simulink model "Project"  (R2017a)
settings: Solver=VariableStepAuto  StartTime=0.0  StopTime=20  FixedStep=0.01  RelTol=1e-3
values from neighbouring files (symbols this model uses):
  b = 2    [initial_condition_and_plots.m]
  c = 4    [initial_condition_and_plots.m]
  C = 2    [initial_condition_and_plots.m]
  Dmax = 3    [initial_condition_and_plots.m]
  init1 = [ -29 -27 pi/6]    [initial_condition_and_plots.m]
  init2 = [ -27 -24 2*pi/3]    [initial_condition_and_plots.m]
  init3 = [ -25 -21 pi/12]    [initial_condition_and_plots.m]
  init4 = [ -23 -19 pi/2]    [initial_condition_and_plots.m]
  init5 = [ -21 -12 5*pi/4]    [initial_condition_and_plots.m]
  K = 4    [initial_condition_and_plots.m]
  K_th = 3    [initial_condition_and_plots.m]
  Kij = 3    [initial_condition_and_plots.m]
  L = 20    [initial_condition_and_plots.m]
  r1k = 3    [initial_condition_and_plots.m]
  r2k = 4    [initial_condition_and_plots.m]
  x1k = 0    [initial_condition_and_plots.m]
  x2k = 15    [initial_condition_and_plots.m]
  y1k = -20    [initial_condition_and_plots.m]
  y2k = -5    [initial_condition_and_plots.m]
  yd = @(i) 4*i-20    [initial_condition_and_plots.m]
(part 1 of 2)
settings Model: Creator=Labis Papakwstas  LastModifiedBy=Labis Papakwstas

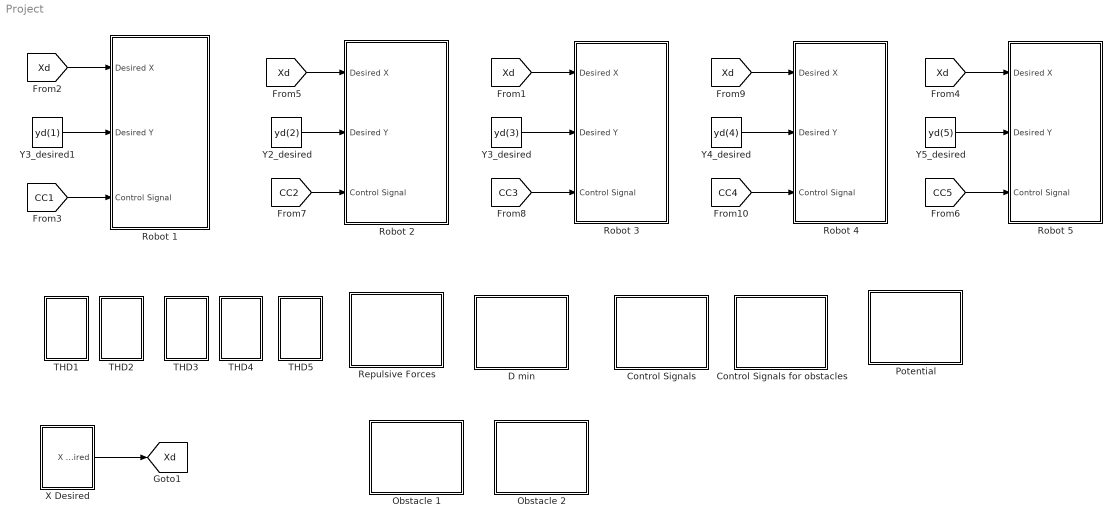
== system Project ==
  "Control Signals " : Subsystem
  Control Signals for obstacles : Subsystem
  D min : Subsystem
  Obstacle 1 : Subsystem
  Obstacle 2 : Subsystem
  Potential : Subsystem
  Repulsive Forces : Subsystem
  "Robot 1 " : Subsystem
  Robot 2 : Subsystem
  Robot 3 : Subsystem
  Robot 4 : Subsystem
  Robot 5 : Subsystem
  "THD1 " : Subsystem
  THD2 : Subsystem
  THD3 : Subsystem
  THD4 : Subsystem
  THD5 : Subsystem
  X Desired : Subsystem
  Y2_desired : Constant  Value=yd(2)
  Y3_desired : Constant  Value=yd(3)
  Y3_desired1 : Constant  Value=yd(1)
  Y4_desired : Constant  Value=yd(4)
  Y5_desired : Constant  Value=yd(5)
  tag scope: Xd=global
  wires:
  [CC3] -> Robot 3/3(Control Signal)
  Y3_desired1/1 -> "Robot 1 "/2("Desired Y ")
  [Xd] -> "Robot 1 "/1(Desired X)
  [CC1] -> "Robot 1 "/3(Control Signal)
  Y2_desired/1 -> Robot 2/2("Desired Y ")
  Y3_desired/1 -> Robot 3/2("Desired Y ")
  [CC2] -> Robot 2/3(Control Signal)
  [Xd] -> Robot 3/1(Desired X)
  X Desired/1(X Desired) -> [Xd]
  [Xd] -> Robot 2/1(Desired X)
  [Xd] -> Robot 5/1(Desired X)
  Y5_desired/1 -> Robot 5/2("Desired Y ")
  [CC5] -> Robot 5/3(Control Signal)
  [CC4] -> Robot 4/3(Control Signal)
  Y4_desired/1 -> Robot 4/2("Desired Y ")
  [Xd] -> Robot 4/1(Desired X)

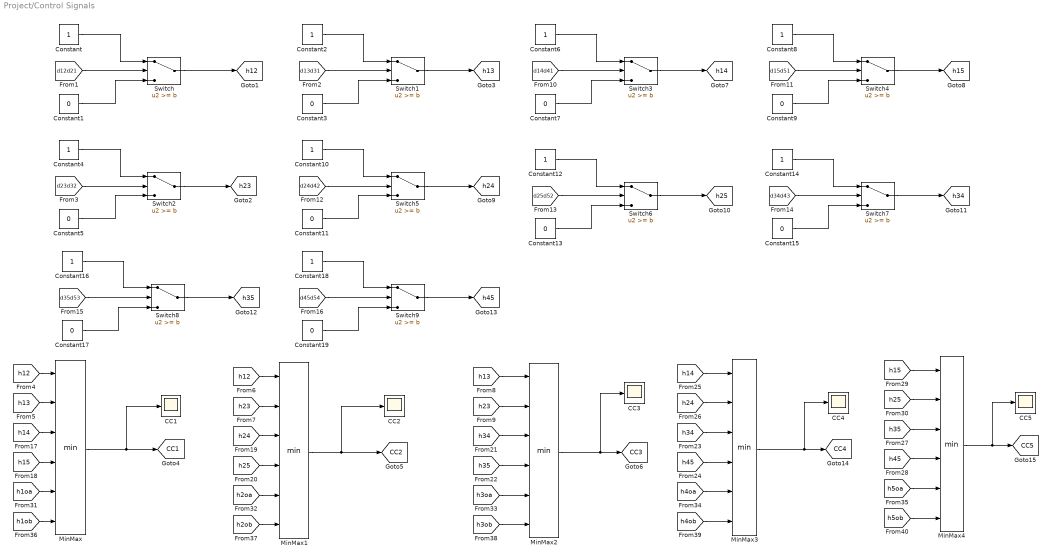
== system Project/Control Signals  ==
  CC1 : Scope
  "CC2 " : Scope
  "CC3 " : Scope
  CC4 : Scope
  CC5 : Scope
  Constant{,2,4,6,8,10,12,14,16,18} (10 alike) : Constant
  Constant{1,3,5,7,9,11,13,15,17,19} (10 alike) : Constant  Value=0
  MinMax{,1..4} (5 alike) : MinMax  Inputs=6
  Switch{,2,5..9} (7 alike) : Switch  Threshold=b
  Switch1 : Switch  Threshold=b  ZeroCross=off
  Switch3 : Switch  Threshold=b  ZeroCross=off
  Switch4 : Switch  Threshold=b  ZeroCross=off
  tag scope: CC1=global, CC2=global, CC3=global, CC4=global, CC5=global, h12=global, h13=global, h14=global, h15=global, h23=global, h24=global, h25=global, h34=global, h35=global, h45=global
  wires:
  [d12d21] -> Switch/2
  Constant/1 -> Switch/1
  Constant1/1 -> Switch/3
  Switch/1 -> [h12]
  [d13d31] -> Switch1/2
  Constant3/1 -> Switch1/3
  Switch1/1 -> [h13]
  Constant2/1 -> Switch1/1
  Switch2/1 -> [h23]
  Constant5/1 -> Switch2/3
  [d23d32] -> Switch2/2
  Constant4/1 -> Switch2/1
  [h12] -> MinMax/1
  [h13] -> MinMax/2
  [h23] -> MinMax1/2
  [h12] -> MinMax1/1
  [h13] -> MinMax2/1
  [h23] -> MinMax2/2
  MinMax1/1 -> "CC2 "/1, [CC2]
  MinMax2/1 -> "CC3 "/1, [CC3]
  MinMax/1 -> CC1/1, [CC1]
  Constant6/1 -> Switch3/1
  Switch3/1 -> [h14]
  Constant7/1 -> Switch3/3
  [d14d41] -> Switch3/2
  [d15d51] -> Switch4/2
  Constant9/1 -> Switch4/3
  Switch4/1 -> [h15]
  Constant8/1 -> Switch4/1
  Constant10/1 -> Switch5/1
  [d24d42] -> Switch5/2
  Constant11/1 -> Switch5/3
  Switch5/1 -> [h24]
  Switch6/1 -> [h25]
  Constant13/1 -> Switch6/3
  [d25d52] -> Switch6/2
  Constant12/1 -> Switch6/1
  Constant14/1 -> Switch7/1
  [d34d43] -> Switch7/2
  Constant15/1 -> Switch7/3
  Switch7/1 -> [h34]
  Switch8/1 -> [h35]
  Constant17/1 -> Switch8/3
  [d35d53] -> Switch8/2
  Constant16/1 -> Switch8/1
  Constant18/1 -> Switch9/1
  [d45d54] -> Switch9/2
  Constant19/1 -> Switch9/3
  Switch9/1 -> [h45]
  [h14] -> MinMax/3
  [h15] -> MinMax/4
  [h24] -> MinMax1/3
  [h25] -> MinMax1/4
  [h34] -> MinMax2/3
  [h35] -> MinMax2/4
  [h45] -> MinMax3/4
  [h34] -> MinMax3/3
  MinMax3/1 -> [CC4], CC4/1
  [h24] -> MinMax3/2
  [h14] -> MinMax3/1
  [h15] -> MinMax4/1
  [h25] -> MinMax4/2
  MinMax4/1 -> [CC5], CC5/1
  [h35] -> MinMax4/3
  [h45] -> MinMax4/4
  [h1oa] -> MinMax/5
  [h2oa] -> MinMax1/5
  [h3oa] -> MinMax2/5
  [h4oa] -> MinMax3/5
  [h5oa] -> MinMax4/5
  [h1ob] -> MinMax/6
  [h2ob] -> MinMax1/6
  [h3ob] -> MinMax2/6
  [h4ob] -> MinMax3/6
  [h5ob] -> MinMax4/6

== system Project/Control Signals for obstacles ==
  Constant{,2,4,6,8,10,12,14,16,18} (10 alike) : Constant
  Constant{1,3,5,7,9,11,13,15,17,19} (10 alike) : Constant  Value=0
  Switch : Switch  Threshold=2  ZeroCross=off
  Switch{1..9} (9 alike) : Switch  Threshold=b
  tag scope: h1oa=global, h1ob=global, h2oa=global, h2ob=global, h3oa=global, h3ob=global, h4oa=global, h4ob=global, h5oa=global, h5ob=global
  wires:
  Switch/1 -> [h1oa]
  Constant1/1 -> Switch/3
  [d1o1] -> Switch/2
  Constant/1 -> Switch/1
  Constant2/1 -> Switch1/1
  [d2o1] -> Switch1/2
  Constant3/1 -> Switch1/3
  Switch1/1 -> [h2oa]
  Switch2/1 -> [h3oa]
  Constant5/1 -> Switch2/3
  [d3o1] -> Switch2/2
  Constant4/1 -> Switch2/1
  Constant6/1 -> Switch3/1
  [d4o1] -> Switch3/2
  Constant7/1 -> Switch3/3
  Switch3/1 -> [h4oa]
  Switch4/1 -> [h5oa]
  Constant9/1 -> Switch4/3
  [d5o1] -> Switch4/2
  Constant8/1 -> Switch4/1
  Constant18/1 -> Switch9/1
  [d5o2] -> Switch9/2
  Constant19/1 -> Switch9/3
  Switch9/1 -> [h5ob]
  Switch8/1 -> [h4ob]
  Constant17/1 -> Switch8/3
  [d4o2] -> Switch8/2
  Constant16/1 -> Switch8/1
  Constant14/1 -> Switch7/1
  [d3o2] -> Switch7/2
  Constant15/1 -> Switch7/3
  Switch7/1 -> [h3ob]
  Switch6/1 -> [h2ob]
  Constant13/1 -> Switch6/3
  [d2o2] -> Switch6/2
  Constant12/1 -> Switch6/1
  Constant10/1 -> Switch5/1
  [d1o2] -> Switch5/2
  Constant11/1 -> Switch5/3
  Switch5/1 -> [h1ob]

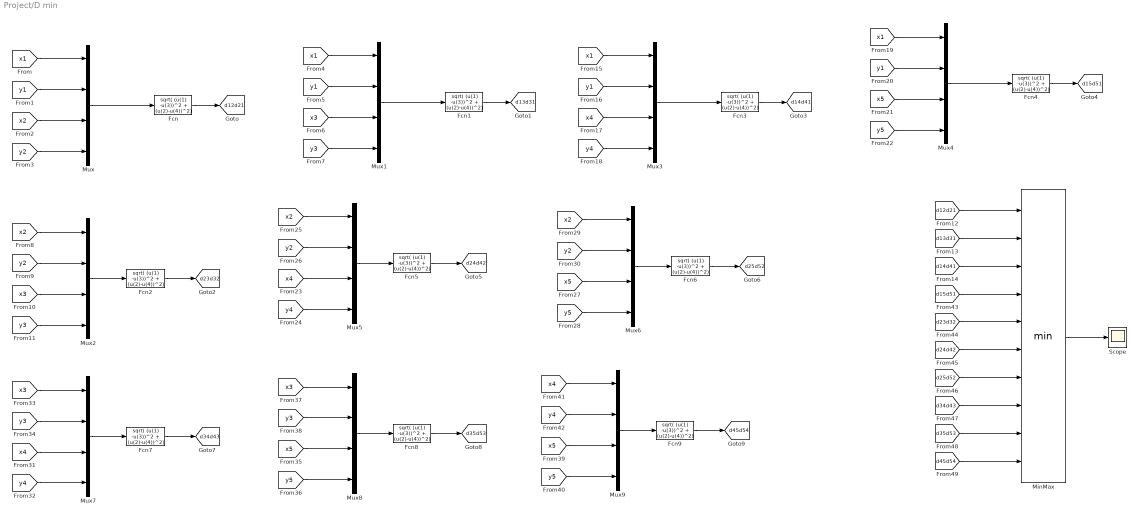
== system Project/D min ==
  Fcn{,1..9} (10 alike) : Fcn  Expr=sqrt( (u(1) -u(3))^2 + (u(2)-u(4))^2)
  MinMax : MinMax  Inputs=10
  Mux{,1..9} (10 alike) : Mux
  Scope : Scope
  tag scope: d12d21=global, d13d31=global, d14d41=global, d15d51=global, d23d32=global, d24d42=global, d25d52=global, d34d43=global, d35d53=global, d45d54=global
  wires:
  [x1] -> Mux/1
  [y1] -> Mux/2
  [x2] -> Mux/3
  [y2] -> Mux/4
  Mux/1 -> Fcn/1
  Mux1/1 -> Fcn1/1
  [y3] -> Mux1/4
  [x3] -> Mux1/3
  [y1] -> Mux1/2
  [x1] -> Mux1/1
  [y2] -> Mux2/2
  [x3] -> Mux2/3
  [x2] -> Mux2/1
  [y3] -> Mux2/4
  Mux2/1 -> Fcn2/1
  Fcn/1 -> [d12d21]
  Fcn1/1 -> [d13d31]
  Fcn2/1 -> [d23d32]
  [d12d21] -> MinMax/1
  [d13d31] -> MinMax/2
  [d14d41] -> MinMax/3
  MinMax/1 -> Scope/1
  Fcn3/1 -> [d14d41]
  [x1] -> Mux3/1
  [y1] -> Mux3/2
  [x4] -> Mux3/3
  [y4] -> Mux3/4
  Mux3/1 -> Fcn3/1
  Mux4/1 -> Fcn4/1
  [y5] -> Mux4/4
  [x5] -> Mux4/3
  [y1] -> Mux4/2
  [x1] -> Mux4/1
  Fcn4/1 -> [d15d51]
  Fcn5/1 -> [d24d42]
  Mux5/1 -> Fcn5/1
  [y4] -> Mux5/4
  [x2] -> Mux5/1
  [x4] -> Mux5/3
  [y2] -> Mux5/2
  [y2] -> Mux6/2
  [x5] -> Mux6/3
  [x2] -> Mux6/1
  [y5] -> Mux6/4
  Mux6/1 -> Fcn6/1
  Fcn6/1 -> [d25d52]
  Fcn7/1 -> [d34d43]
  Mux7/1 -> Fcn7/1
  [y4] -> Mux7/4
  [x3] -> Mux7/1
  [x4] -> Mux7/3
  [y3] -> Mux7/2
  [y3] -> Mux8/2
  [x5] -> Mux8/3
  [x3] -> Mux8/1
  [y5] -> Mux8/4
  Mux8/1 -> Fcn8/1
  Fcn8/1 -> [d35d53]
  Fcn9/1 -> [d45d54]
  Mux9/1 -> Fcn9/1
  [y5] -> Mux9/4
  [x4] -> Mux9/1
  [x5] -> Mux9/3
  [y4] -> Mux9/2
  [d15d51] -> MinMax/4
  [d23d32] -> MinMax/5
  [d24d42] -> MinMax/6
  [d25d52] -> MinMax/7
  [d34d43] -> MinMax/8
  [d35d53] -> MinMax/9
  [d45d54] -> MinMax/10

== system Project/Obstacle 1 ==
  Constant{,3,6,9,12} (5 alike) : Constant  Value=x1k
  Constant{1,4,7,10,13} (5 alike) : Constant  Value=y1k
  Constant{2,5,8,11,14} (5 alike) : Constant  Value=r1k
  Fcn : Fcn  Expr="u(5)*u(1)/(sqrt( (u(1) - u(2))^2 + (u(3) - u(4))^2)) +u(2)* ( 1 - (u(5)/sqrt( ( u(1) - u(2) )^2 + ( u(3) - u(4) )^2) )  )"
  Fcn1 : Fcn  Expr=u(5)*u(3)/(sqrt( (u(1) - u(2))^2 + (u(3) - u(4))^2)) + ( 1 - (u(5)/sqrt( (u(1) - u(2))^2 + (u(3) - u(4))^2)) )*u(4)
  Fcn{2,4,6,8} (4 alike) : Fcn  Expr=u(5)*u(1)/(sqrt( (u(1) - u(2))^2 + (u(3) - u(4))^2)) + ( 1 - u(5)/(sqrt( (u(1) - u(2))^2 + (u(3) - u(4))^2)) )*u(2)
  Fcn{3,5,7,9} (4 alike) : Fcn  Expr=u(5)*u(3)/(sqrt( (u(1) - u(2))^2 + (u(3) - u(4))^2)) + ( 1 - u(5)/(sqrt( (u(1) - u(2))^2 + (u(3) - u(4))^2)) )*u(4)
  Mux{,1..4} (5 alike) : Mux  Inputs=5
  "Obstacle Distance " : Subsystem
  tag scope: x1o1=global, x2o1=global, x3o1=global, x4o1=global, x5o1=global, y1o1=global, y2o1=global, y3o1=global, y4o1=global, y5o1=global
  wires:
  [x1] -> Mux/1
  [y1] -> Mux/3
  Constant2/1 -> Mux/5
  Constant1/1 -> Mux/4
  Constant/1 -> Mux/2
  Mux/1 -> Fcn1/1, Fcn/1
  Fcn/1 -> [x1o1]
  Fcn1/1 -> [y1o1]
  Fcn3/1 -> [y2o1]
  [y2] -> Mux1/3
  [x2] -> Mux1/1
  Constant5/1 -> Mux1/5
  Constant3/1 -> Mux1/2
  Constant4/1 -> Mux1/4
  Fcn2/1 -> [x2o1]
  Mux1/1 -> Fcn3/1, Fcn2/1
  Mux2/1 -> Fcn5/1, Fcn4/1
  Fcn4/1 -> [x3o1]
  Constant6/1 -> Mux2/2
  [x3] -> Mux2/1
  Constant8/1 -> Mux2/5
  [y3] -> Mux2/3
  Constant7/1 -> Mux2/4
  Fcn5/1 -> [y3o1]
  Fcn7/1 -> [y4o1]
  Constant10/1 -> Mux3/4
  [y4] -> Mux3/3
  Constant11/1 -> Mux3/5
  [x4] -> Mux3/1
  Constant9/1 -> Mux3/2
  Fcn6/1 -> [x4o1]
  Mux3/1 -> Fcn6/1, Fcn7/1
  Mux4/1 -> Fcn8/1, Fcn9/1
  Fcn8/1 -> [x5o1]
  Constant13/1 -> Mux4/4
  Constant12/1 -> Mux4/2
  Constant14/1 -> Mux4/5
  [x5] -> Mux4/1
  [y5] -> Mux4/3
  Fcn9/1 -> [y5o1]

== system Project/Obstacle 2 ==
  Constant{,3,6,9,12} (5 alike) : Constant  Value=x2k
  Constant{1,4,7,10,13} (5 alike) : Constant  Value=y2k
  Constant{2,5,8,11,14} (5 alike) : Constant  Value=r2k
  Fcn : Fcn  Expr="u(5)*u(1)/(sqrt( (u(1) - u(2))^2 + (u(3) - u(4))^2)) +u(2)* ( 1 - (u(5)/sqrt( ( u(1) - u(2) )^2 + ( u(3) - u(4) )^2) )  )"
  Fcn1 : Fcn  Expr=u(5)*u(3)/(sqrt( (u(1) - u(2))^2 + (u(3) - u(4))^2)) + ( 1 - (u(5)/sqrt( (u(1) - u(2))^2 + (u(3) - u(4))^2)) )*u(4)
  Fcn{2,4,6,8} (4 alike) : Fcn  Expr=u(5)*u(1)/(sqrt( (u(1) - u(2))^2 + (u(3) - u(4))^2)) + ( 1 - u(5)/(sqrt( (u(1) - u(2))^2 + (u(3) - u(4))^2)) )*u(2)
  Fcn{3,5,7,9} (4 alike) : Fcn  Expr=u(5)*u(3)/(sqrt( (u(1) - u(2))^2 + (u(3) - u(4))^2)) + ( 1 - u(5)/(sqrt( (u(1) - u(2))^2 + (u(3) - u(4))^2)) )*u(4)
  Mux{,1..4} (5 alike) : Mux  Inputs=5
  "Obstacle Distance " : Subsystem
  tag scope: x1o2=global, x2o2=global, x3o2=global, x4o2=global, x5o2=global, y1o2=global, y2o2=global, y3o2=global, y4o2=global, y5o2=global
  wires:
  Fcn9/1 -> [y5o2]
  [y5] -> Mux4/3
  [x5] -> Mux4/1
  Constant14/1 -> Mux4/5
  Constant12/1 -> Mux4/2
  Constant13/1 -> Mux4/4
  Fcn8/1 -> [x5o2]
  Mux4/1 -> Fcn9/1, Fcn8/1
  Mux3/1 -> Fcn7/1, Fcn6/1
  Fcn6/1 -> [x4o2]
  Constant9/1 -> Mux3/2
  [x4] -> Mux3/1
  Constant11/1 -> Mux3/5
  [y4] -> Mux3/3
  Constant10/1 -> Mux3/4
  Fcn7/1 -> [y4o2]
  Fcn5/1 -> [y3o2]
  Constant7/1 -> Mux2/4
  [y3] -> Mux2/3
  Constant8/1 -> Mux2/5
  [x3] -> Mux2/1
  Constant6/1 -> Mux2/2
  Fcn4/1 -> [x3o2]
  Mux2/1 -> Fcn4/1, Fcn5/1
  Mux1/1 -> Fcn2/1, Fcn3/1
  Fcn2/1 -> [x2o2]
  Constant4/1 -> Mux1/4
  Constant3/1 -> Mux1/2
  Constant5/1 -> Mux1/5
  [x2] -> Mux1/1
  [y2] -> Mux1/3
  Fcn3/1 -> [y2o2]
  Fcn1/1 -> [y1o2]
  Fcn/1 -> [x1o2]
  Mux/1 -> Fcn/1, Fcn1/1
  Constant/1 -> Mux/2
  Constant1/1 -> Mux/4
  Constant2/1 -> Mux/5
  [y1] -> Mux/3
  [x1] -> Mux/1

== system Project/Potential ==
  Sum : Sum  Inputs=|+++++
  VA1 : Subsystem
  VA2 : Subsystem
  VA3 : Subsystem
  VA4 : Subsystem
  VA5 : Subsystem
  Va : Scope
  tag scope: Va1=global, Va2=global, Va3=global, Va4=global, Va5=global
  wires:
  VA1/1(Vi) -> [Va1]
  VA2/1(Vi) -> [Va2]
  [Va1] -> Sum/1
  [Va2] -> Sum/2
  [Va3] -> Sum/3
  Sum/1 -> Va/1
  VA3/1(Vi) -> [Va3]
  VA4/1(Vi) -> [Va4]
  VA5/1(Vi) -> [Va5]
  [Va5] -> Sum/5
  [Va4] -> Sum/4

== system Project/Repulsive Forces ==
  Forces Robot1 : Subsystem
  Forces Robot2 : Subsystem
  Forces Robot3 : Subsystem
  Forces Robot4 : Subsystem
  Forces Robot5 : Subsystem
  tag scope: F1x=global, F1y=global, F2x=global, F2y=global, F3x=global, F3y=global, F4x=global, F4y=global, F5x=global, F5y=global
  wires:
  Forces Robot3/1(Fx) -> [F3x]
  Forces Robot3/2(Fy) -> [F3y]
  Forces Robot4/2(Fy) -> [F4y]
  Forces Robot4/1(Fx) -> [F4x]
  Forces Robot5/1(Fx) -> [F5x]
  Forces Robot5/2(Fy) -> [F5y]
  Forces Robot1/1(Fx) -> [F1x]
  Forces Robot1/2(Fy) -> [F1y]
  Forces Robot2/1(Fx) -> [F2x]
  Forces Robot2/2(Fy) -> [F2y]

== system Project/Robot 1  ==
  Desired X : Inport
  "Desired Y " : Inport  Port=2
  Control Signal : Inport  Port=3
  Fcn1 : Fcn  Expr=sqrt( u(1) ^2 + u(2)^2)
  Mux1 : Mux  Inputs=2
  TH1 : Scope
  Tracking Control : Subsystem
  U1 : Scope
  V1 : Scope
  X1 : Scope
  Y1 : Scope
  tag scope: th1=global, x1=global, y1=global
  wires:
  [th1] -> Tracking Control/5(TH1)
  [y1] -> Tracking Control/3(Y1)
  [x1] -> Tracking Control/1(X1)
  Tracking Control/5("U ") -> U1/1
  Tracking Control/4(V) -> V1/1
  Tracking Control/3("TH ") -> TH1/1, [th1]
  Tracking Control/2(Y) -> Y1/1, [y1]
  Tracking Control/1(X) -> X1/1, [x1]
  "Desired Y "/1 -> Tracking Control/4(Yd)
  Desired X/1 -> Tracking Control/2(Xd)
  [F1x] -> Mux1/2
  Mux1/1 -> Fcn1/1
  [F1y] -> Mux1/1
  Fcn1/1 -> Tracking Control/7(Dc)
  Control Signal/1 -> Tracking Control/8(CC)
  [thd1] -> Tracking Control/6(THc)

== system Project/Robot 2 ==
  Desired X : Inport
  "Desired Y " : Inport  Port=2
  Control Signal : Inport  Port=3
  Fcn1 : Fcn  Expr=sqrt( u(1) ^2 + u(2)^2)
  Mux1 : Mux  Inputs=2
  TH2 : Scope
  Tracking Control1 : Subsystem
  U2 : Scope
  V2 : Scope
  X2 : Scope
  Y2 : Scope
  tag scope: th2=global, x2=global, y2=global
  wires:
  Fcn1/1 -> Tracking Control1/7(Dc)
  Control Signal/1 -> Tracking Control1/8(CC)
  Tracking Control1/4(V) -> V2/1
  Tracking Control1/5("U ") -> U2/1
  Mux1/1 -> Fcn1/1
  [thd2] -> Tracking Control1/6(THc)
  [F2x] -> Mux1/2
  Desired X/1 -> Tracking Control1/2(Xd)
  [th2] -> Tracking Control1/5(TH1)
  [x2] -> Tracking Control1/1(X1)
  "Desired Y "/1 -> Tracking Control1/4(Yd)
  Tracking Control1/2(Y) -> Y2/1, [y2]
  Tracking Control1/1(X) -> X2/1, [x2]
  Tracking Control1/3("TH ") -> TH2/1, [th2]
  [F2y] -> Mux1/1
  [y2] -> Tracking Control1/3(Y1)

== system Project/Robot 3 ==
  Desired X : Inport
  "Desired Y " : Inport  Port=2
  Control Signal : Inport  Port=3
  Fcn1 : Fcn  Expr=sqrt( u(1) ^2 + u(2)^2)
  Mux1 : Mux  Inputs=2
  TH3 : Scope
  Tracking Control : Subsystem
  U3 : Scope
  V3 : Scope
  "X3 " : Scope
  Y3 : Scope
  tag scope: th3=global, x3=global, y3=global
  wires:
  [F3y] -> Mux1/1
  Tracking Control/2(Y) -> Y3/1, [y3]
  Desired X/1 -> Tracking Control/2(Xd)
  [th3] -> Tracking Control/5(TH1)
  [x3] -> Tracking Control/1(X1)
  "Desired Y "/1 -> Tracking Control/4(Yd)
  Mux1/1 -> Fcn1/1
  Control Signal/1 -> Tracking Control/8(CC)
  Fcn1/1 -> Tracking Control/7(Dc)
  Tracking Control/4(V) -> V3/1
  [thd3] -> Tracking Control/6(THc)
  [F3x] -> Mux1/2
  [y3] -> Tracking Control/3(Y1)
  Tracking Control/3("TH ") -> TH3/1, [th3]
  Tracking Control/1(X) -> "X3 "/1, [x3]
  Tracking Control/5("U ") -> U3/1

== system Project/Robot 4 ==
  Desired X : Inport
  "Desired Y " : Inport  Port=2
  Control Signal : Inport  Port=3
  Fcn1 : Fcn  Expr=sqrt( u(1) ^2 + u(2)^2)
  Mux1 : Mux  Inputs=2
  "TH4 " : Scope
  Tracking Control : Subsystem
  U4 : Scope
  V4 : Scope
  "X4 " : Scope
  Y4 : Scope
  tag scope: th4=global, x4=global, y4=global
  wires:
  [F4y] -> Mux1/1
  Tracking Control/2(Y) -> Y4/1, [y4]
  Desired X/1 -> Tracking Control/2(Xd)
  [th4] -> Tracking Control/5(TH1)
  [x4] -> Tracking Control/1(X1)
  "Desired Y "/1 -> Tracking Control/4(Yd)
  Mux1/1 -> Fcn1/1
  Control Signal/1 -> Tracking Control/8(CC)
  Fcn1/1 -> Tracking Control/7(Dc)
  Tracking Control/4(V) -> V4/1
  [thd4] -> Tracking Control/6(THc)
  [F4x] -> Mux1/2
  [y4] -> Tracking Control/3(Y1)
  Tracking Control/3("TH ") -> "TH4 "/1, [th4]
  Tracking Control/1(X) -> "X4 "/1, [x4]
  Tracking Control/5("U ") -> U4/1

== system Project/Robot 5 ==
  Desired X : Inport
  "Desired Y " : Inport  Port=2
  Control Signal : Inport  Port=3
  Fcn1 : Fcn  Expr=sqrt( u(1) ^2 + u(2)^2)
  Mux1 : Mux  Inputs=2
  TH5 : Scope
  Tracking Control : Subsystem
  U5 : Scope
  V5 : Scope
  "X5 " : Scope
  Y5 : Scope
  tag scope: th5=global, x5=global, y5=global
  wires:
  Tracking Control/5("U ") -> U5/1
  Tracking Control/1(X) -> [x5], "X5 "/1
  Tracking Control/3("TH ") -> [th5], TH5/1
  [y5] -> Tracking Control/3(Y1)
  [F5x] -> Mux1/2
  [thd5] -> Tracking Control/6(THc)
  Tracking Control/4(V) -> V5/1
  Fcn1/1 -> Tracking Control/7(Dc)
  Control Signal/1 -> Tracking Control/8(CC)
  Mux1/1 -> Fcn1/1
  "Desired Y "/1 -> Tracking Control/4(Yd)
  [x5] -> Tracking Control/1(X1)
  [th5] -> Tracking Control/5(TH1)
  Desired X/1 -> Tracking Control/2(Xd)
  Tracking Control/2(Y) -> [y5], Y5/1
  [F5y] -> Mux1/1

== system Project/THD1  ==
  Fcn3 : Fcn  Expr=atan2(-u(1),-u(2))
  Mux3 : Mux  Inputs=2
  Switch1 : Switch  Criteria=u2 ~= 0  ZeroCross=off
  Switch2 : Switch  Criteria=u2 ~= 0  ZeroCross=off
  THD for obstacle 1 : Subsystem
  THD for obstacle 2 : Subsystem
  tag scope: thd1=global, thd1f=global
  wires:
  [thd1oa] -> Switch1/3
  [thd1f] -> Switch1/1
  [h1oa] -> Switch1/2
  Mux3/1 -> Fcn3/1
  [F1x] -> Mux3/2
  [F1y] -> Mux3/1
  Fcn3/1 -> [thd1f]
  [h1ob] -> Switch2/2
  [thd1ob] -> Switch2/3
  Switch1/1 -> Switch2/1
  Switch2/1 -> [thd1]

== system Project/THD2 ==
  Fcn3 : Fcn  Expr=atan2(-u(1),-u(2))
  Mux3 : Mux  Inputs=2
  Switch1 : Switch  Criteria=u2 ~= 0  ZeroCross=off
  Switch2 : Switch  Criteria=u2 ~= 0  ZeroCross=off
  THD for obstacle 1 : Subsystem
  THD for obstacle 2 : Subsystem
  tag scope: thd2=global, thd2f=global
  wires:
  Switch2/1 -> [thd2]
  [F2x] -> Mux3/2
  Fcn3/1 -> [thd2f]
  Mux3/1 -> Fcn3/1
  [F2y] -> Mux3/1
  [h2oa] -> Switch1/2
  [thd2oa] -> Switch1/3
  [h2ob] -> Switch2/2
  Switch1/1 -> Switch2/1
  [thd2ob] -> Switch2/3
  [thd2f] -> Switch1/1

== system Project/THD3 ==
  Fcn3 : Fcn  Expr=atan2(-u(1),-u(2))
  Mux3 : Mux  Inputs=2
  Switch1 : Switch  Criteria=u2 ~= 0  ZeroCross=off
  Switch2 : Switch  Criteria=u2 ~= 0  ZeroCross=off
  THD for obstacle 1 : Subsystem
  THD for obstacle 2 : Subsystem
  tag scope: thd3=global, thd3f=global
  wires:
  Switch2/1 -> [thd3]
  [F3x] -> Mux3/2
  Fcn3/1 -> [thd3f]
  Mux3/1 -> Fcn3/1
  [F3y] -> Mux3/1
  [h3oa] -> Switch1/2
  [thd3oa] -> Switch1/3
  [h3ob] -> Switch2/2
  Switch1/1 -> Switch2/1
  [thd3ob] -> Switch2/3
  [thd3f] -> Switch1/1

== system Project/THD4 ==
  Fcn3 : Fcn  Expr=atan2(-u(1),-u(2))
  Mux3 : Mux  Inputs=2
  Switch1 : Switch  Criteria=u2 ~= 0  ZeroCross=off
  Switch2 : Switch  Criteria=u2 ~= 0  ZeroCross=off
  THD for obstacle 1 : Subsystem
  THD for obstacle 2 : Subsystem
  tag scope: thd4=global, thd4f=global
  wires:
  Switch2/1 -> [thd4]
  [F4x] -> Mux3/2
  Fcn3/1 -> [thd4f]
  Mux3/1 -> Fcn3/1
  [F4y] -> Mux3/1
  [h4oa] -> Switch1/2
  [thd4oa] -> Switch1/3
  [h4ob] -> Switch2/2
  Switch1/1 -> Switch2/1
  [thd4ob] -> Switch2/3
  [thd4f] -> Switch1/1

== system Project/THD5 ==
  Fcn3 : Fcn  Expr=atan2(-u(1),-u(2))
  Mux3 : Mux  Inputs=2
  Switch1 : Switch  Criteria=u2 ~= 0  ZeroCross=off
  Switch2 : Switch  Criteria=u2 ~= 0  ZeroCross=off
  THD for obstacle 1 : Subsystem
  THD for obstacle 2 : Subsystem
  tag scope: thd5=global, thd5f=global
  wires:
  Switch2/1 -> [thd5]
  [F5x] -> Mux3/2
  Fcn3/1 -> [thd5f]
  Mux3/1 -> Fcn3/1
  [F5y] -> Mux3/1
  [h5oa] -> Switch1/2
  [thd5oa] -> Switch1/3
  [h5ob] -> Switch2/2
  Switch1/1 -> Switch2/1
  [thd5ob] -> Switch2/3
  [thd5f] -> Switch1/1

== system Project/X Desired ==
  Clock : Clock
  Product : Product
  Scope7 : Scope
  Sum5 : Sum  Inputs=|++
  "X_desired " : Constant  Value=L
  X_desired 2 : Constant  Value=C
  X Desired : Outport
  wires:
  Clock/1 -> Product/1
  "X_desired "/1 -> Sum5/1
  X_desired 2/1 -> Product/2
  Product/1 -> Sum5/2
  Sum5/1 -> X Desired/1, Scope7/1

== system Project/Obstacle 1/Obstacle Distance  ==
  Fcn{1..5} (5 alike) : Fcn  Expr=sqrt( (u(1) -u(3))^2 + (u(2)-u(4))^2)
  Mux{1..5} (5 alike) : Mux
  tag scope: d1o1=global, d2o1=global, d3o1=global, d4o1=global, d5o1=global
  wires:
  [x1o1] -> Mux3/3
  Mux3/1 -> Fcn3/1
  [y1] -> Mux3/2
  Fcn3/1 -> [d1o1]
  [y1o1] -> Mux3/4
  [x1] -> Mux3/1
  [x2] -> Mux1/1
  [y2o1] -> Mux1/4
  Fcn1/1 -> [d2o1]
  [y2] -> Mux1/2
  Mux1/1 -> Fcn1/1
  [x2o1] -> Mux1/3
  [x3o1] -> Mux2/3
  Mux2/1 -> Fcn2/1
  [y3] -> Mux2/2
  Fcn2/1 -> [d3o1]
  [y3o1] -> Mux2/4
  [x3] -> Mux2/1
  [x4] -> Mux4/1
  [y4o1] -> Mux4/4
  Fcn4/1 -> [d4o1]
  [y4] -> Mux4/2
  Mux4/1 -> Fcn4/1
  [x4o1] -> Mux4/3
  [x5o1] -> Mux5/3
  Mux5/1 -> Fcn5/1
  [y5] -> Mux5/2
  Fcn5/1 -> [d5o1]
  [y5o1] -> Mux5/4
  [x5] -> Mux5/1

== system Project/Obstacle 2/Obstacle Distance  ==
  Fcn{1..5} (5 alike) : Fcn  Expr=sqrt( (u(1) -u(3))^2 + (u(2)-u(4))^2)
  Mux{1..5} (5 alike) : Mux
  tag scope: d1o2=global, d2o2=global, d3o2=global, d4o2=global, d5o2=global
  wires:
  [x5] -> Mux5/1
  [y5o2] -> Mux5/4
  Fcn5/1 -> [d5o2]
  [y5] -> Mux5/2
  Mux5/1 -> Fcn5/1
  [x5o2] -> Mux5/3
  [x4o2] -> Mux4/3
  Mux4/1 -> Fcn4/1
  [y4] -> Mux4/2
  Fcn4/1 -> [d4o2]
  [y4o2] -> Mux4/4
  [x4] -> Mux4/1
  [x3] -> Mux2/1
  [y3o2] -> Mux2/4
  Fcn2/1 -> [d3o2]
  [y3] -> Mux2/2
  Mux2/1 -> Fcn2/1
  [x3o2] -> Mux2/3
  [x2o2] -> Mux1/3
  Mux1/1 -> Fcn1/1
  [y2] -> Mux1/2
  Fcn1/1 -> [d2o2]
  [y2o2] -> Mux1/4
  [x2] -> Mux1/1
  [x1] -> Mux3/1
  [y1o2] -> Mux3/4
  Fcn3/1 -> [d1o2]
  [y1] -> Mux3/2
  Mux3/1 -> Fcn3/1
  [x1o2] -> Mux3/3

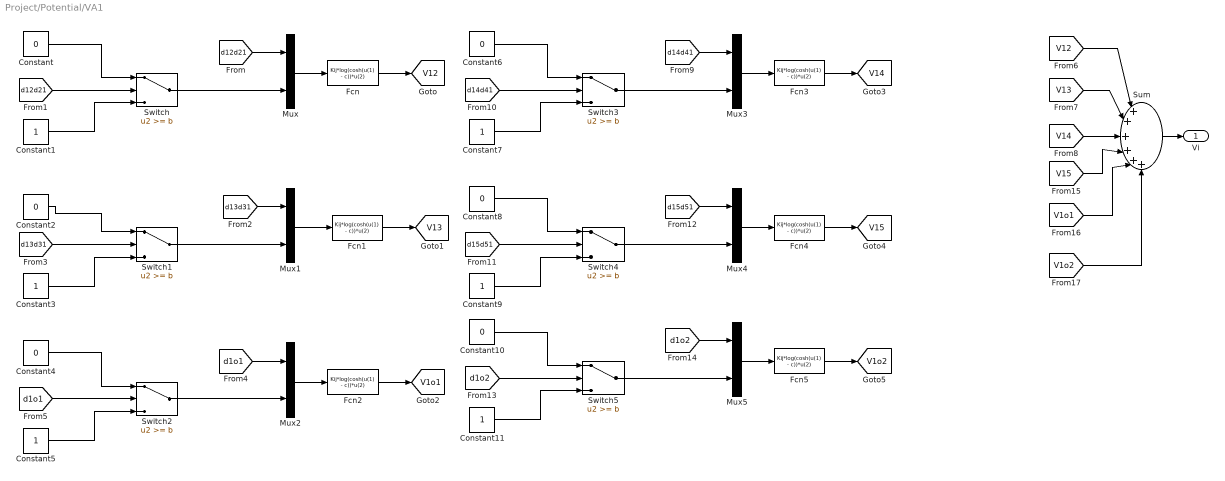
== system Project/Potential/VA1 ==
  Constant{,2,4,6,8,10} (6 alike) : Constant  Value=0
  Constant{1,3,5,7,9,11} (6 alike) : Constant
  Fcn{,1..5} (6 alike) : Fcn  Expr=Kij*log(cosh(u(1) - c))*u(2)
  Mux{,1..5} (6 alike) : Mux  Inputs=2
  Sum : Sum  Inputs=|++++++
  Switch{,1..5} (6 alike) : Switch  Threshold=b
  Vi : Outport
  tag scope: V12=global, V13=global, V14=global, V15=global, V1o1=global, V1o2=global
  wires:
  Fcn/1 -> [V12]
  Mux/1 -> Fcn/1
  Mux2/1 -> Fcn2/1
  [d1o1] -> Mux2/1
  Fcn2/1 -> [V1o1]
  [V12] -> Sum/1
  [d12d21] -> Mux/1
  [V13] -> Sum/2
  Sum/1 -> Vi/1
  Mux1/1 -> Fcn1/1
  [d13d31] -> Mux1/1
  Fcn1/1 -> [V13]
  [V14] -> Sum/3
  Constant/1 -> Switch/1
  Constant1/1 -> Switch/3
  [d12d21] -> Switch/2
  Switch/1 -> Mux/2
  [d13d31] -> Switch1/2
  Constant3/1 -> Switch1/3
  Constant2/1 -> Switch1/1
  Constant4/1 -> Switch2/1
  Constant5/1 -> Switch2/3
  [d1o1] -> Switch2/2
  Switch1/1 -> Mux1/2
  Switch2/1 -> Mux2/2
  Switch3/1 -> Mux3/2
  [d14d41] -> Switch3/2
  Constant7/1 -> Switch3/3
  Constant6/1 -> Switch3/1
  [d14d41] -> Mux3/1
  Mux3/1 -> Fcn3/1
  Fcn3/1 -> [V14]
  Fcn4/1 -> [V15]
  Mux4/1 -> Fcn4/1
  [d15d51] -> Mux4/1
  Constant8/1 -> Switch4/1
  Constant9/1 -> Switch4/3
  [d15d51] -> Switch4/2
  Switch4/1 -> Mux4/2
  Switch5/1 -> Mux5/2
  [d1o2] -> Switch5/2
  Constant11/1 -> Switch5/3
  Constant10/1 -> Switch5/1
  [d1o2] -> Mux5/1
  Mux5/1 -> Fcn5/1
  Fcn5/1 -> [V1o2]
  [V15] -> Sum/4
  [V1o1] -> Sum/5
  [V1o2] -> Sum/6

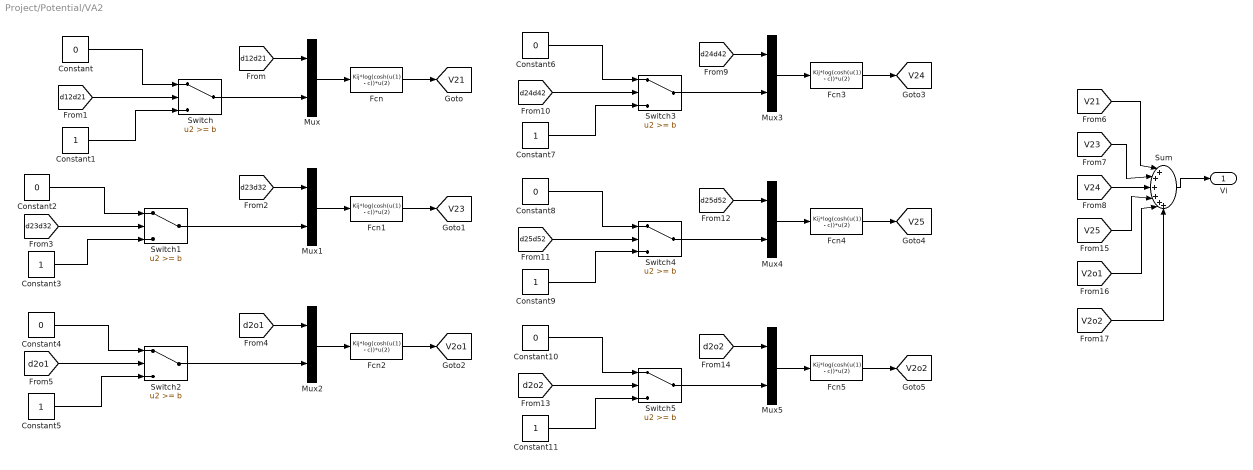
== system Project/Potential/VA2 ==
  Constant{,2,4,6,8,10} (6 alike) : Constant  Value=0
  Constant{1,3,5,7,9,11} (6 alike) : Constant
  Fcn{,1..5} (6 alike) : Fcn  Expr=Kij*log(cosh(u(1) - c))*u(2)
  Mux{,1..5} (6 alike) : Mux  Inputs=2
  Sum : Sum  Inputs=|++++++
  Switch{,1..5} (6 alike) : Switch  Threshold=b
  Vi : Outport
  tag scope: V21=global, V23=global, V24=global, V25=global, V2o1=global, V2o2=global
  wires:
  Fcn1/1 -> [V23]
  [d23d32] -> Mux1/1
  Mux1/1 -> Fcn1/1
  Sum/1 -> Vi/1
  [V23] -> Sum/2
  [d12d21] -> Mux/1
  [V21] -> Sum/1
  Fcn2/1 -> [V2o1]
  [d2o1] -> Mux2/1
  Mux2/1 -> Fcn2/1
  Mux/1 -> Fcn/1
  Fcn/1 -> [V21]
  [V24] -> Sum/3
  Constant/1 -> Switch/1
  Constant1/1 -> Switch/3
  [d12d21] -> Switch/2
  Switch/1 -> Mux/2
  Constant2/1 -> Switch1/1
  Constant3/1 -> Switch1/3
  [d23d32] -> Switch1/2
  Switch1/1 -> Mux1/2
  [d2o1] -> Switch2/2
  Constant5/1 -> Switch2/3
  Constant4/1 -> Switch2/1
  Switch2/1 -> Mux2/2
  Switch3/1 -> Mux3/2
  [d24d42] -> Switch3/2
  Constant7/1 -> Switch3/3
  Constant6/1 -> Switch3/1
  Fcn3/1 -> [V24]
  Mux3/1 -> Fcn3/1
  [d24d42] -> Mux3/1
  [d25d52] -> Mux4/1
  Mux4/1 -> Fcn4/1
  Fcn4/1 -> [V25]
  Constant8/1 -> Switch4/1
  Constant9/1 -> Switch4/3
  [d25d52] -> Switch4/2
  Switch4/1 -> Mux4/2
  Switch5/1 -> Mux5/2
  [d2o2] -> Switch5/2
  Constant11/1 -> Switch5/3
  Constant10/1 -> Switch5/1
  Fcn5/1 -> [V2o2]
  Mux5/1 -> Fcn5/1
  [d2o2] -> Mux5/1
  [V25] -> Sum/4
  [V2o1] -> Sum/5
  [V2o2] -> Sum/6

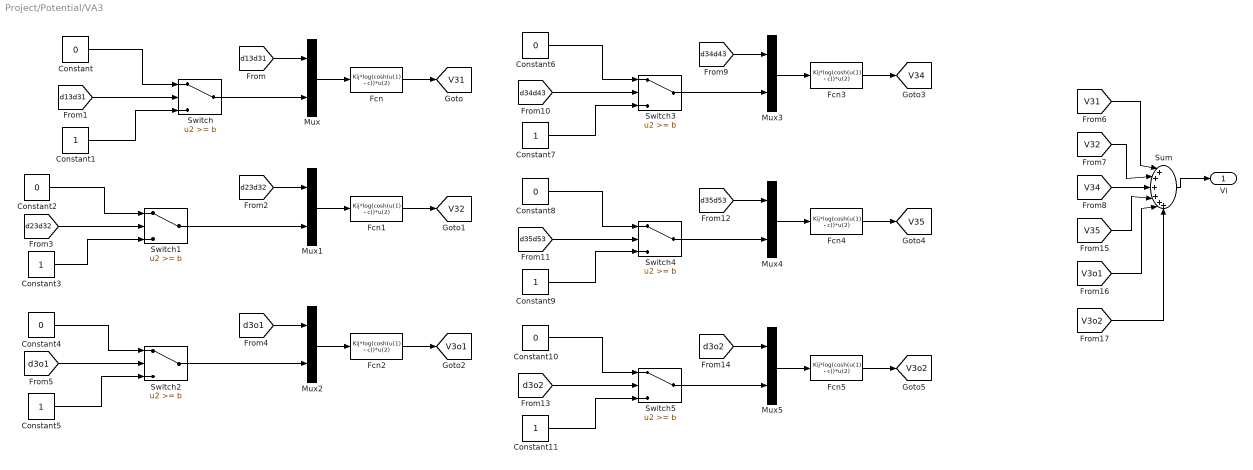
== system Project/Potential/VA3 ==
  Constant{,2,4,6,8,10} (6 alike) : Constant  Value=0
  Constant{1,3,5,7,9,11} (6 alike) : Constant
  Fcn{,1..5} (6 alike) : Fcn  Expr=Kij*log(cosh(u(1) - c))*u(2)
  Mux{,1..5} (6 alike) : Mux  Inputs=2
  Sum : Sum  Inputs=|++++++
  Switch{,1..5} (6 alike) : Switch  Threshold=b
  Vi : Outport
  tag scope: V31=global, V32=global, V34=global, V35=global, V3o1=global, V3o2=global
  wires:
  [V3o2] -> Sum/6
  [V3o1] -> Sum/5
  [V35] -> Sum/4
  [d3o2] -> Mux5/1
  Mux5/1 -> Fcn5/1
  Fcn5/1 -> [V3o2]
  Constant10/1 -> Switch5/1
  Constant11/1 -> Switch5/3
  [d3o2] -> Switch5/2
  Switch5/1 -> Mux5/2
  Switch4/1 -> Mux4/2
  [d35d53] -> Switch4/2
  Constant9/1 -> Switch4/3
  Constant8/1 -> Switch4/1
  Fcn4/1 -> [V35]
  Mux4/1 -> Fcn4/1
  [d35d53] -> Mux4/1
  [d34d43] -> Mux3/1
  Mux3/1 -> Fcn3/1
  Fcn3/1 -> [V34]
  Constant6/1 -> Switch3/1
  Constant7/1 -> Switch3/3
  [d34d43] -> Switch3/2
  Switch3/1 -> Mux3/2
  Switch2/1 -> Mux2/2
  Constant4/1 -> Switch2/1
  Constant5/1 -> Switch2/3
  [d3o1] -> Switch2/2
  Switch1/1 -> Mux1/2
  [d23d32] -> Switch1/2
  Constant3/1 -> Switch1/3
  Constant2/1 -> Switch1/1
  Switch/1 -> Mux/2
  [d13d31] -> Switch/2
  Constant1/1 -> Switch/3
  Constant/1 -> Switch/1
  [V34] -> Sum/3
  Fcn/1 -> [V31]
  Mux/1 -> Fcn/1
  Mux2/1 -> Fcn2/1
  [d3o1] -> Mux2/1
  Fcn2/1 -> [V3o1]
  [V31] -> Sum/1
  [d13d31] -> Mux/1
  [V32] -> Sum/2
  Sum/1 -> Vi/1
  Mux1/1 -> Fcn1/1
  [d23d32] -> Mux1/1
  Fcn1/1 -> [V32]

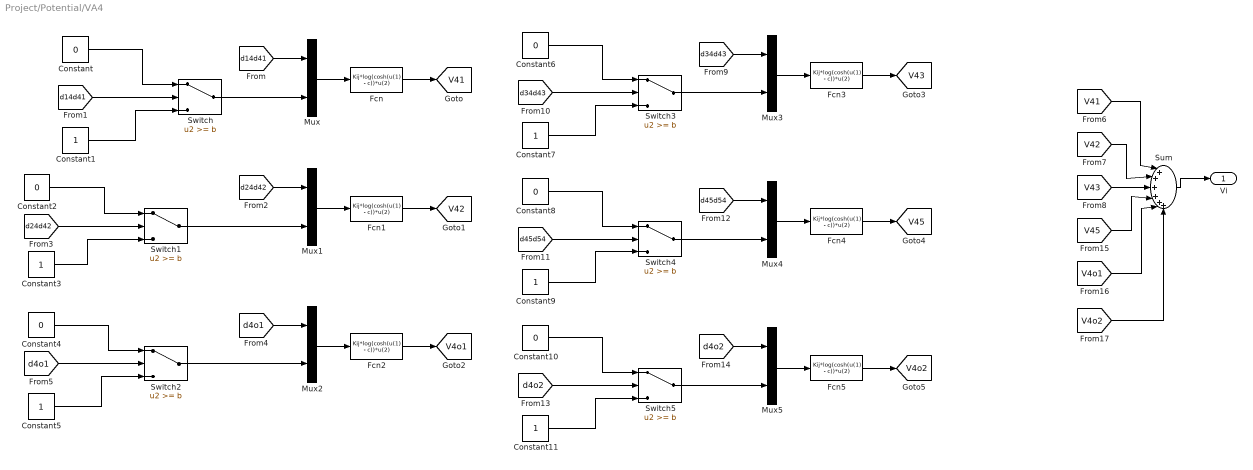
== system Project/Potential/VA4 ==
  Constant{,2,4,6,8,10} (6 alike) : Constant  Value=0
  Constant{1,3,5,7,9,11} (6 alike) : Constant
  Fcn{,1..5} (6 alike) : Fcn  Expr=Kij*log(cosh(u(1) - c))*u(2)
  Mux{,1..5} (6 alike) : Mux  Inputs=2
  Sum : Sum  Inputs=|++++++
  Switch{,1..5} (6 alike) : Switch  Threshold=b
  Vi : Outport
  tag scope: V41=global, V42=global, V43=global, V45=global, V4o1=global, V4o2=global
  wires:
  Fcn1/1 -> [V42]
  [d24d42] -> Mux1/1
  Mux1/1 -> Fcn1/1
  Sum/1 -> Vi/1
  [V42] -> Sum/2
  [d14d41] -> Mux/1
  [V41] -> Sum/1
  Fcn2/1 -> [V4o1]
  [d4o1] -> Mux2/1
  Mux2/1 -> Fcn2/1
  Mux/1 -> Fcn/1
  Fcn/1 -> [V41]
  [V43] -> Sum/3
  Constant/1 -> Switch/1
  Constant1/1 -> Switch/3
  [d14d41] -> Switch/2
  Switch/1 -> Mux/2
  Constant2/1 -> Switch1/1
  Constant3/1 -> Switch1/3
  [d24d42] -> Switch1/2
  Switch1/1 -> Mux1/2
  [d4o1] -> Switch2/2
  Constant5/1 -> Switch2/3
  Constant4/1 -> Switch2/1
  Switch2/1 -> Mux2/2
  Switch3/1 -> Mux3/2
  [d34d43] -> Switch3/2
  Constant7/1 -> Switch3/3
  Constant6/1 -> Switch3/1
  Fcn3/1 -> [V43]
  Mux3/1 -> Fcn3/1
  [d34d43] -> Mux3/1
  [d45d54] -> Mux4/1
  Mux4/1 -> Fcn4/1
  Fcn4/1 -> [V45]
  Constant8/1 -> Switch4/1
  Constant9/1 -> Switch4/3
  [d45d54] -> Switch4/2
  Switch4/1 -> Mux4/2
  Switch5/1 -> Mux5/2
  [d4o2] -> Switch5/2
  Constant11/1 -> Switch5/3
  Constant10/1 -> Switch5/1
  Fcn5/1 -> [V4o2]
  Mux5/1 -> Fcn5/1
  [d4o2] -> Mux5/1
  [V45] -> Sum/4
  [V4o1] -> Sum/5
  [V4o2] -> Sum/6

== system Project/Potential/VA5 ==
  Constant{,2,4,6,8,10} (6 alike) : Constant  Value=0
  Constant{1,3,5,7,9,11} (6 alike) : Constant
  Fcn{,1..5} (6 alike) : Fcn  Expr=Kij*log(cosh(u(1) - c))*u(2)
  Mux{,1..5} (6 alike) : Mux  Inputs=2
  Sum : Sum  Inputs=|++++++
  Switch{,1..5} (6 alike) : Switch  Threshold=b
  Vi : Outport
  tag scope: V51=global, V52=global, V53=global, V54=global, V5o1=global, V5o2=global
  wires:
  [V5o2] -> Sum/6
  [V5o1] -> Sum/5
  [V54] -> Sum/4
  [d5o2] -> Mux5/1
  Mux5/1 -> Fcn5/1
  Fcn5/1 -> [V5o2]
  Constant10/1 -> Switch5/1
  Constant11/1 -> Switch5/3
  [d5o2] -> Switch5/2
  Switch5/1 -> Mux5/2
  Switch4/1 -> Mux4/2
  [d45d54] -> Switch4/2
  Constant9/1 -> Switch4/3
  Constant8/1 -> Switch4/1
  Fcn4/1 -> [V54]
  Mux4/1 -> Fcn4/1
  [d45d54] -> Mux4/1
  [d35d53] -> Mux3/1
  Mux3/1 -> Fcn3/1
  Fcn3/1 -> [V53]
  Constant6/1 -> Switch3/1
  Constant7/1 -> Switch3/3
  [d35d53] -> Switch3/2
  Switch3/1 -> Mux3/2
  Switch2/1 -> Mux2/2
  Constant4/1 -> Switch2/1
  Constant5/1 -> Switch2/3
  [d5o1] -> Switch2/2
  Switch1/1 -> Mux1/2
  [d25d52] -> Switch1/2
  Constant3/1 -> Switch1/3
  Constant2/1 -> Switch1/1
  Switch/1 -> Mux/2
  [d15d51] -> Switch/2
  Constant1/1 -> Switch/3
  Constant/1 -> Switch/1
  [V53] -> Sum/3
  Fcn/1 -> [V51]
  Mux/1 -> Fcn/1
  Mux2/1 -> Fcn2/1
  [d5o1] -> Mux2/1
  Fcn2/1 -> [V5o1]
  [V51] -> Sum/1
  [d15d51] -> Mux/1
  [V52] -> Sum/2
  Sum/1 -> Vi/1
  Mux1/1 -> Fcn1/1
  [d25d52] -> Mux1/1
  Fcn1/1 -> [V52]

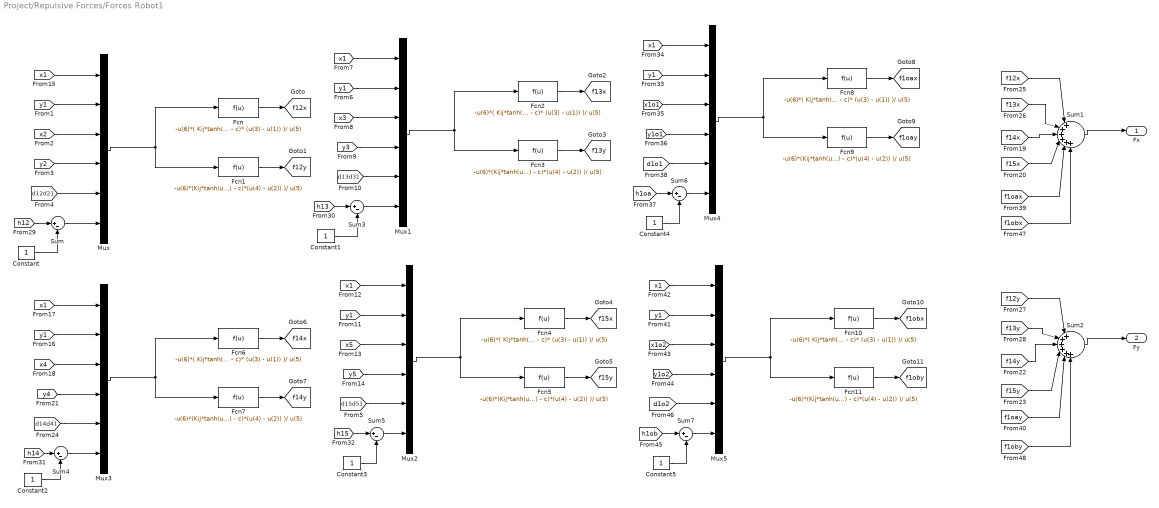
== system Project/Repulsive Forces/Forces Robot1 ==
  Constant{,1..5} (6 alike) : Constant
  Fcn{,2,4,6,8,10} (6 alike) : Fcn  Expr=-u(6)*( Kij*tanh(u(5) - c)* (u(3) - u(1)) )/ u(5)
  Fcn{1,3,5,7,9,11} (6 alike) : Fcn  Expr=-u(6)*(Kij*tanh(u(5) - c)*(u(4) - u(2)) )/ u(5)
  Mux{,1..5} (6 alike) : Mux  Inputs=6
  Sum{,3..7} (6 alike) : Sum  Inputs=|+-
  Sum1 : Sum  Inputs=|++++++
  Sum2 : Sum  Inputs=|++++++
  Fx : Outport
  Fy : Outport  Port=2
  tag scope: f12x=global, f12y=global, f13x=global, f13y=global, f14x=global, f14y=global, f15x=global, f15y=global, f1oax=global, f1oay=global, f1obx=global, f1oby=global
  wires:
  Mux/1 -> Fcn1/1, Fcn/1
  [y2] -> Mux/4
  [x1] -> Mux/1
  Fcn1/1 -> [f12y]
  Fcn/1 -> [f12x]
  [x2] -> Mux/3
  [y1] -> Mux/2
  [x3] -> Mux1/3
  [y1] -> Mux1/2
  Fcn3/1 -> [f13y]
  Mux1/1 -> Fcn3/1, Fcn2/1
  Fcn2/1 -> [f13x]
  [d13d31] -> Mux1/5
  [y3] -> Mux1/4
  [x1] -> Mux1/1
  [d12d21] -> Mux/5
  [x1] -> Mux2/1
  [y5] -> Mux2/4
  [d15d51] -> Mux2/5
  Fcn4/1 -> [f15x]
  Mux2/1 -> Fcn4/1, Fcn5/1
  Fcn5/1 -> [f15y]
  [y1] -> Mux2/2
  [x5] -> Mux2/3
  [x4] -> Mux3/3
  [y1] -> Mux3/2
  Fcn7/1 -> [f14y]
  Mux3/1 -> Fcn7/1, Fcn6/1
  Fcn6/1 -> [f14x]
  [d14d41] -> Mux3/5
  [y4] -> Mux3/4
  [x1] -> Mux3/1
  Sum2/1 -> Fy/1
  [f13y] -> Sum2/2
  [f12y] -> Sum2/1
  Sum1/1 -> Fx/1
  [f13x] -> Sum1/2
  [f12x] -> Sum1/1
  [f14x] -> Sum1/3
  [f15x] -> Sum1/4
  [f14y] -> Sum2/3
  [f15y] -> Sum2/4
  [h12] -> Sum/1
  Sum/1 -> Mux/6
  Constant/1 -> Sum/2
  Constant1/1 -> Sum3/2
  Sum3/1 -> Mux1/6
  [h13] -> Sum3/1
  Constant2/1 -> Sum4/2
  [h14] -> Sum4/1
  Sum4/1 -> Mux3/6
  Constant3/1 -> Sum5/2
  [h15] -> Sum5/1
  Sum5/1 -> Mux2/6
  Sum6/1 -> Mux4/6
  [h1oa] -> Sum6/1
  Constant4/1 -> Sum6/2
  [x1o1] -> Mux4/3
  [y1] -> Mux4/2
  Fcn9/1 -> [f1oay]
  Mux4/1 -> Fcn9/1, Fcn8/1
  Fcn8/1 -> [f1oax]
  [d1o1] -> Mux4/5
  [y1o1] -> Mux4/4
  [x1] -> Mux4/1
  [f1oax] -> Sum1/5
  [f1oay] -> Sum2/5
  [x1] -> Mux5/1
  [y1o2] -> Mux5/4
  [d1o2] -> Mux5/5
  Fcn10/1 -> [f1obx]
  Mux5/1 -> Fcn10/1, Fcn11/1
  Fcn11/1 -> [f1oby]
  [y1] -> Mux5/2
  [x1o2] -> Mux5/3
  Constant5/1 -> Sum7/2
  [h1ob] -> Sum7/1
  Sum7/1 -> Mux5/6
  [f1obx] -> Sum1/6
  [f1oby] -> Sum2/6

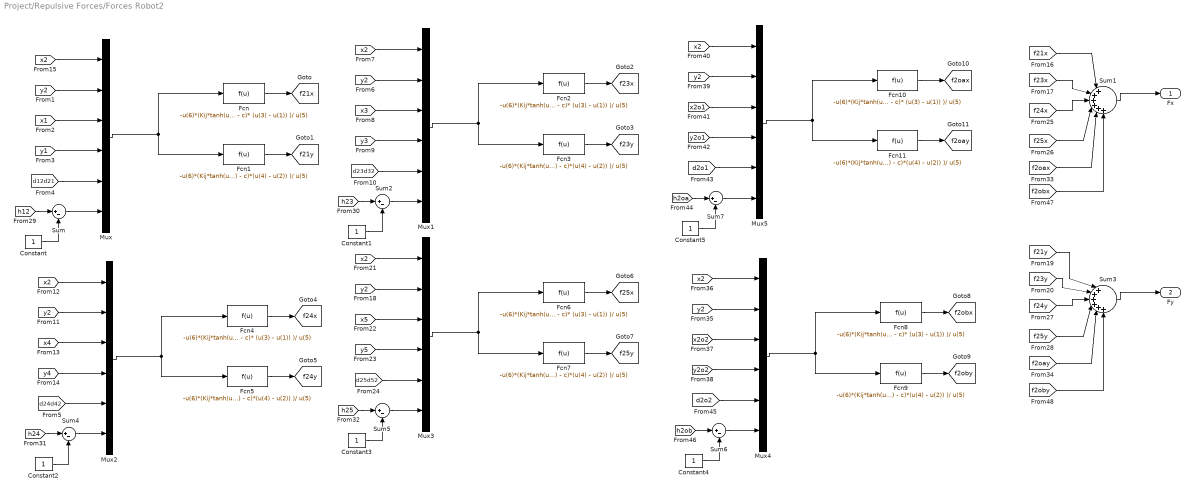
== system Project/Repulsive Forces/Forces Robot2 ==
  Constant{,1..5} (6 alike) : Constant
  Fcn{,2,4,6,8,10} (6 alike) : Fcn  Expr=-u(6)*(Kij*tanh(u(5) - c)* (u(3) - u(1)) )/ u(5)
  Fcn{1,3,5,7,9,11} (6 alike) : Fcn  Expr=-u(6)*(Kij*tanh(u(5) - c)*(u(4) - u(2)) )/ u(5)
  Mux{,1..5} (6 alike) : Mux  Inputs=6
  Sum{,2,4..7} (6 alike) : Sum  Inputs=|+-
  Sum1 : Sum  Inputs=|++++++
  Sum3 : Sum  Inputs=|++++++
  Fx : Outport
  Fy : Outport  Port=2
  tag scope: f21x=global, f21y=global, f23x=global, f23y=global, f24x=global, f24y=global, f25x=global, f25y=global, f2oax=global, f2oay=global, f2obx=global, f2oby=global
  wires:
  [d12d21] -> Mux/5
  Mux1/1 -> Fcn2/1, Fcn3/1
  [x2] -> Mux1/1
  [y3] -> Mux1/4
  [d23d32] -> Mux1/5
  Fcn2/1 -> [f23x]
  Fcn3/1 -> [f23y]
  [y2] -> Mux1/2
  [x3] -> Mux1/3
  [y2] -> Mux/2
  [x1] -> Mux/3
  Fcn/1 -> [f21x]
  Fcn1/1 -> [f21y]
  [x2] -> Mux/1
  [y1] -> Mux/4
  Mux/1 -> Fcn1/1, Fcn/1
  [x4] -> Mux2/3
  [y2] -> Mux2/2
  Fcn5/1 -> [f24y]
  Fcn4/1 -> [f24x]
  [d24d42] -> Mux2/5
  [y4] -> Mux2/4
  [x2] -> Mux2/1
  Mux2/1 -> Fcn5/1, Fcn4/1
  [f21x] -> Sum1/1
  [f23x] -> Sum1/2
  Sum1/1 -> Fx/1
  Sum3/1 -> Fy/1
  [f23y] -> Sum3/2
  [f21y] -> Sum3/1
  Mux3/1 -> Fcn6/1, Fcn7/1
  [x2] -> Mux3/1
  [y5] -> Mux3/4
  [d25d52] -> Mux3/5
  Fcn6/1 -> [f25x]
  Fcn7/1 -> [f25y]
  [y2] -> Mux3/2
  [x5] -> Mux3/3
  [f24x] -> Sum1/3
  [f25x] -> Sum1/4
  [f24y] -> Sum3/3
  [f25y] -> Sum3/4
  Constant/1 -> Sum/2
  Sum/1 -> Mux/6
  [h12] -> Sum/1
  Constant1/1 -> Sum2/2
  Sum2/1 -> Mux1/6
  [h23] -> Sum2/1
  Constant2/1 -> Sum4/2
  [h24] -> Sum4/1
  Sum4/1 -> Mux2/6
  Constant3/1 -> Sum5/2
  Sum5/1 -> Mux3/6
  [h25] -> Sum5/1
  Mux5/1 -> Fcn10/1, Fcn11/1
  [x2] -> Mux5/1
  [y2o1] -> Mux5/4
  [d2o1] -> Mux5/5
  Fcn10/1 -> [f2oax]
  Fcn11/1 -> [f2oay]
  [y2] -> Mux5/2
  [x2o1] -> Mux5/3
  Constant5/1 -> Sum7/2
  Sum7/1 -> Mux5/6
  [h2oa] -> Sum7/1
  [f2oax] -> Sum1/5
  [f2oay] -> Sum3/5
  [h2ob] -> Sum6/1
  Sum6/1 -> Mux4/6
  Constant4/1 -> Sum6/2
  [x2o2] -> Mux4/3
  [y2] -> Mux4/2
  Fcn9/1 -> [f2oby]
  Fcn8/1 -> [f2obx]
  [d2o2] -> Mux4/5
  [y2o2] -> Mux4/4
  [x2] -> Mux4/1
  Mux4/1 -> Fcn9/1, Fcn8/1
  [f2obx] -> Sum1/6
  [f2oby] -> Sum3/6

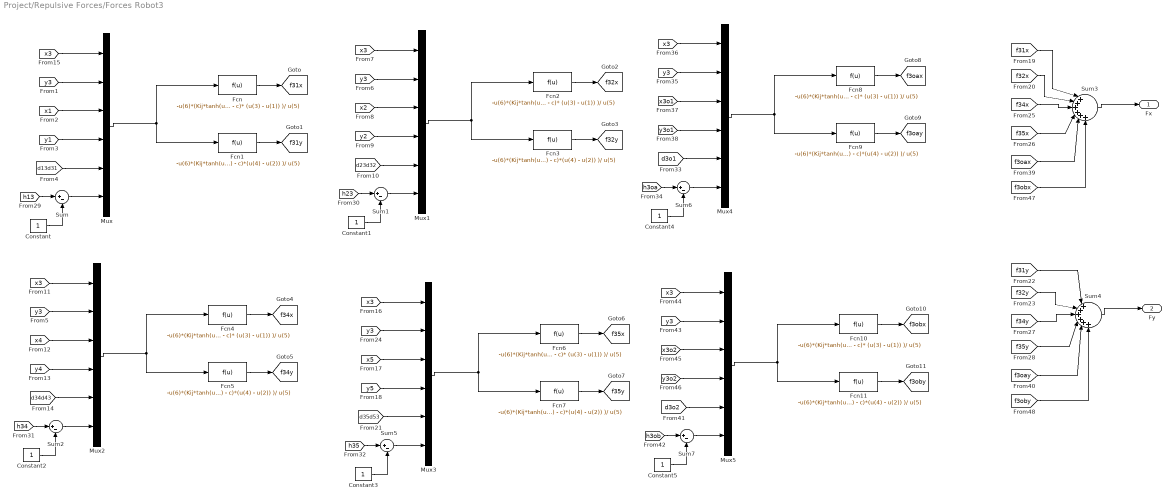
== system Project/Repulsive Forces/Forces Robot3 ==
  Constant{,1..5} (6 alike) : Constant
  Fcn{,2,4,6,8,10} (6 alike) : Fcn  Expr=-u(6)*(Kij*tanh(u(5) - c)* (u(3) - u(1)) )/ u(5)
  Fcn{1,3,5,7,9,11} (6 alike) : Fcn  Expr=-u(6)*(Kij*tanh(u(5) - c)*(u(4) - u(2)) )/ u(5)
  Mux{,1..5} (6 alike) : Mux  Inputs=6
  Sum{,1..2,5..7} (6 alike) : Sum  Inputs=|+-
  Sum3 : Sum  Inputs=|++++++
  Sum4 : Sum  Inputs=|++++++
  Fx : Outport
  Fy : Outport  Port=2
  tag scope: f31x=global, f31y=global, f32x=global, f32y=global, f34x=global, f34y=global, f35x=global, f35y=global, f3oax=global, f3oay=global, f3obx=global, f3oby=global
  wires:
  Mux/1 -> Fcn1/1, Fcn/1
  [y1] -> Mux/4
  [x3] -> Mux/1
  [f31x] -> Sum3/1
  Fcn1/1 -> [f31y]
  [f32x] -> Sum3/2
  Fcn/1 -> [f31x]
  [x1] -> Mux/3
  [y3] -> Mux/2
  Sum3/1 -> Fx/1
  [x2] -> Mux1/3
  [y3] -> Mux1/2
  Fcn3/1 -> [f32y]
  Mux1/1 -> Fcn3/1, Fcn2/1
  Fcn2/1 -> [f32x]
  [d23d32] -> Mux1/5
  [y2] -> Mux1/4
  [x3] -> Mux1/1
  [d13d31] -> Mux/5
  [f31y] -> Sum4/1
  [f32y] -> Sum4/2
  Sum4/1 -> Fy/1
  [d34d43] -> Mux2/5
  [y3] -> Mux2/2
  [x4] -> Mux2/3
  Fcn4/1 -> [f34x]
  Fcn5/1 -> [f34y]
  [x3] -> Mux2/1
  [y4] -> Mux2/4
  Mux2/1 -> Fcn4/1, Fcn5/1
  Mux3/1 -> Fcn7/1, Fcn6/1
  [y5] -> Mux3/4
  Fcn7/1 -> [f35y]
  Fcn6/1 -> [f35x]
  [x5] -> Mux3/3
  [y3] -> Mux3/2
  [d35d53] -> Mux3/5
  [x3] -> Mux3/1
  [f34x] -> Sum3/3
  [f35x] -> Sum3/4
  [f34y] -> Sum4/3
  [f35y] -> Sum4/4
  Constant/1 -> Sum/2
  Sum/1 -> Mux/6
  [h13] -> Sum/1
  Constant1/1 -> Sum1/2
  Sum1/1 -> Mux1/6
  [h23] -> Sum1/1
  Constant2/1 -> Sum2/2
  Sum2/1 -> Mux2/6
  [h34] -> Sum2/1
  Constant3/1 -> Sum5/2
  Sum5/1 -> Mux3/6
  [h35] -> Sum5/1
  [h3oa] -> Sum6/1
  Sum6/1 -> Mux4/6
  Constant4/1 -> Sum6/2
  [x3] -> Mux4/1
  [y3o1] -> Mux4/4
  [d3o1] -> Mux4/5
  Fcn8/1 -> [f3oax]
  Mux4/1 -> Fcn8/1, Fcn9/1
  Fcn9/1 -> [f3oay]
  [y3] -> Mux4/2
  [x3o1] -> Mux4/3
  [f3oax] -> Sum3/5
  [f3oay] -> Sum4/5
  [x3o2] -> Mux5/3
  [y3] -> Mux5/2
  Fcn11/1 -> [f3oby]
  Mux5/1 -> Fcn11/1, Fcn10/1
  Fcn10/1 -> [f3obx]
  [d3o2] -> Mux5/5
  [y3o2] -> Mux5/4
  [x3] -> Mux5/1
  Constant5/1 -> Sum7/2
  Sum7/1 -> Mux5/6
  [h3ob] -> Sum7/1
  [f3obx] -> Sum3/6
  [f3oby] -> Sum4/6

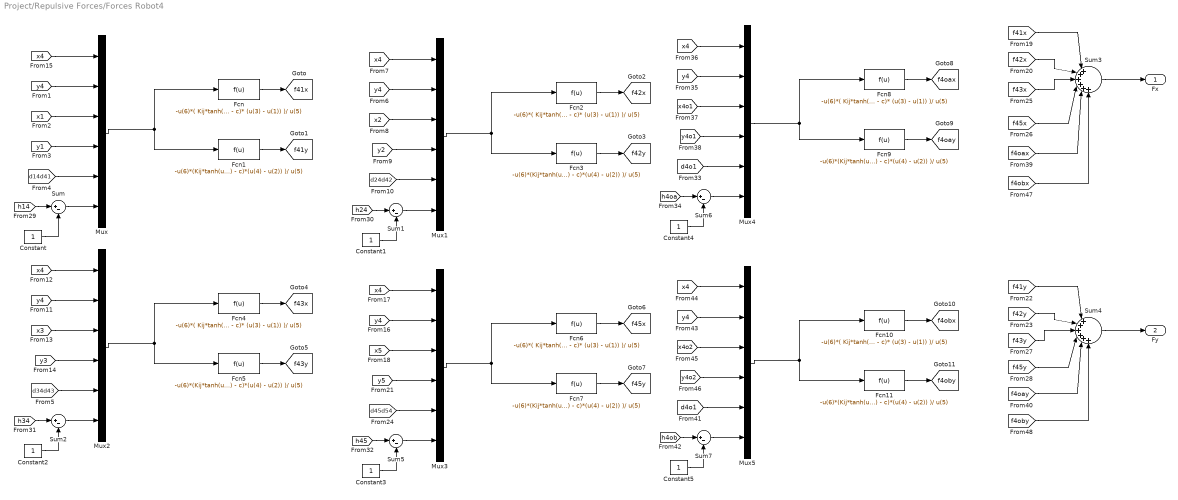
== system Project/Repulsive Forces/Forces Robot4 ==
  Constant{,1..5} (6 alike) : Constant
  Fcn{,2,4,6,8,10} (6 alike) : Fcn  Expr=-u(6)*( Kij*tanh(u(5) - c)* (u(3) - u(1)) )/ u(5)
  Fcn{1,3,5,7,9,11} (6 alike) : Fcn  Expr=-u(6)*(Kij*tanh(u(5) - c)*(u(4) - u(2)) )/ u(5)
  Mux{,1..5} (6 alike) : Mux  Inputs=6
  Sum{,1..2,5..7} (6 alike) : Sum  Inputs=|+-
  Sum3 : Sum  Inputs=|++++++
  Sum4 : Sum  Inputs=|++++++
  Fx : Outport
  Fy : Outport  Port=2
  tag scope: f41x=global, f41y=global, f42x=global, f42y=global, f43x=global, f43y=global, f45x=global, f45y=global, f4oax=global, f4oay=global, f4obx=global, f4oby=global
  wires:
  Sum4/1 -> Fy/1
  [f42y] -> Sum4/2
  [f41y] -> Sum4/1
  [d14d41] -> Mux/5
  [x4] -> Mux1/1
  [y2] -> Mux1/4
  [d24d42] -> Mux1/5
  Fcn2/1 -> [f42x]
  Mux1/1 -> Fcn2/1, Fcn3/1
  Fcn3/1 -> [f42y]
  [y4] -> Mux1/2
  [x2] -> Mux1/3
  Sum3/1 -> Fx/1
  [y4] -> Mux/2
  [x1] -> Mux/3
  Fcn/1 -> [f41x]
  [f42x] -> Sum3/2
  Fcn1/1 -> [f41y]
  [f41x] -> Sum3/1
  [x4] -> Mux/1
  [y1] -> Mux/4
  Mux/1 -> Fcn/1, Fcn1/1
  [x3] -> Mux2/3
  [y4] -> Mux2/2
  Fcn5/1 -> [f43y]
  Mux2/1 -> Fcn5/1, Fcn4/1
  Fcn4/1 -> [f43x]
  [d34d43] -> Mux2/5
  [y3] -> Mux2/4
  [x4] -> Mux2/1
  [x4] -> Mux3/1
  [y5] -> Mux3/4
  [d45d54] -> Mux3/5
  Fcn6/1 -> [f45x]
  Mux3/1 -> Fcn6/1, Fcn7/1
  Fcn7/1 -> [f45y]
  [y4] -> Mux3/2
  [x5] -> Mux3/3
  [f43x] -> Sum3/3
  [f45x] -> Sum3/4
  [f43y] -> Sum4/3
  [f45y] -> Sum4/4
  Constant/1 -> Sum/2
  Sum/1 -> Mux/6
  [h14] -> Sum/1
  Constant1/1 -> Sum1/2
  Sum1/1 -> Mux1/6
  [h24] -> Sum1/1
  Constant2/1 -> Sum2/2
  Sum2/1 -> Mux2/6
  [h34] -> Sum2/1
  Constant3/1 -> Sum5/2
  Sum5/1 -> Mux3/6
  [h45] -> Sum5/1
  [h4oa] -> Sum6/1
  Sum6/1 -> Mux4/6
  Constant4/1 -> Sum6/2
  [x4o1] -> Mux4/3
  [y4] -> Mux4/2
  Fcn9/1 -> [f4oay]
  Mux4/1 -> Fcn8/1, Fcn9/1
  Fcn8/1 -> [f4oax]
  [d4o1] -> Mux4/5
  [y4o1] -> Mux4/4
  [x4] -> Mux4/1
  [f4oax] -> Sum3/5
  [f4oay] -> Sum4/5
  [x4] -> Mux5/1
  [y4o2] -> Mux5/4
  [d4o1] -> Mux5/5
  Fcn10/1 -> [f4obx]
  Mux5/1 -> Fcn10/1, Fcn11/1
  Fcn11/1 -> [f4oby]
  [y4] -> Mux5/2
  [x4o2] -> Mux5/3
  Constant5/1 -> Sum7/2
  Sum7/1 -> Mux5/6
  [h4ob] -> Sum7/1
  [f4obx] -> Sum3/6
  [f4oby] -> Sum4/6

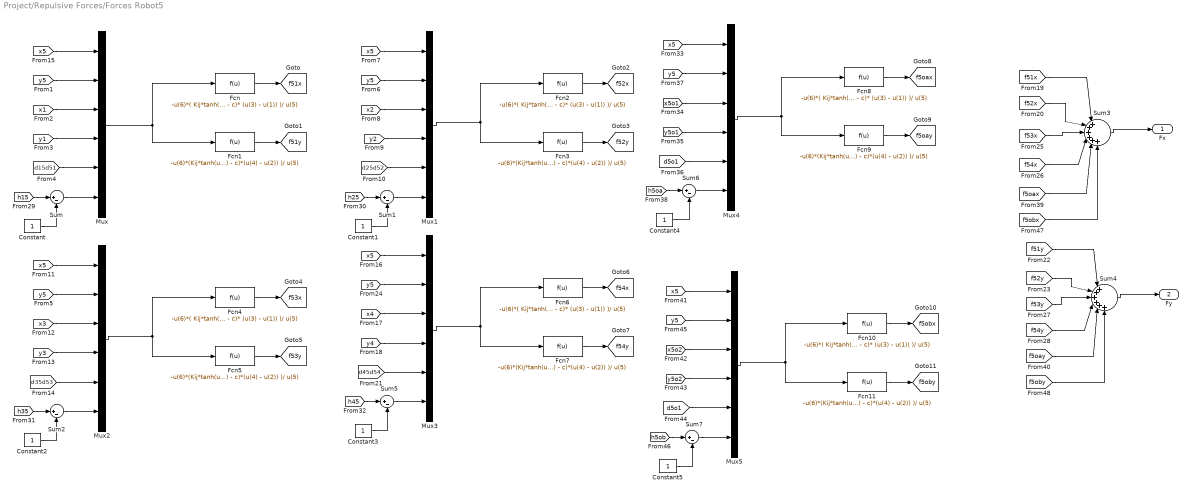
== system Project/Repulsive Forces/Forces Robot5 ==
  Constant{,1..5} (6 alike) : Constant
  Fcn{,2,4,6,8,10} (6 alike) : Fcn  Expr=-u(6)*( Kij*tanh(u(5) - c)* (u(3) - u(1)) )/ u(5)
  Fcn{1,3,5,7,9,11} (6 alike) : Fcn  Expr=-u(6)*(Kij*tanh(u(5) - c)*(u(4) - u(2)) )/ u(5)
  Mux{,1..5} (6 alike) : Mux  Inputs=6
  Sum{,1..2,5..7} (6 alike) : Sum  Inputs=|+-
  Sum3 : Sum  Inputs=|++++++
  Sum4 : Sum  Inputs=|++++++
  Fx : Outport
  Fy : Outport  Port=2
  tag scope: f51x=global, f51y=global, f52x=global, f52y=global, f53x=global, f53y=global, f54x=global, f54y=global, f5oax=global, f5oay=global, f5obx=global, f5oby=global
  wires:
  Mux/1 -> Fcn/1, Fcn1/1
  [y1] -> Mux/4
  [x5] -> Mux/1
  [f51x] -> Sum3/1
  Fcn1/1 -> [f51y]
  [f52x] -> Sum3/2
  Fcn/1 -> [f51x]
  [x1] -> Mux/3
  [y5] -> Mux/2
  Sum3/1 -> Fx/1
  [x2] -> Mux1/3
  [y5] -> Mux1/2
  Fcn3/1 -> [f52y]
  Mux1/1 -> Fcn3/1, Fcn2/1
  Fcn2/1 -> [f52x]
  [d25d52] -> Mux1/5
  [y2] -> Mux1/4
  [x5] -> Mux1/1
  [d15d51] -> Mux/5
  [f51y] -> Sum4/1
  [f52y] -> Sum4/2
  Sum4/1 -> Fy/1
  [d35d53] -> Mux2/5
  [y5] -> Mux2/2
  [x3] -> Mux2/3
  Fcn4/1 -> [f53x]
  Fcn5/1 -> [f53y]
  [x5] -> Mux2/1
  [y3] -> Mux2/4
  Mux2/1 -> Fcn4/1, Fcn5/1
  Mux3/1 -> Fcn7/1, Fcn6/1
  [y4] -> Mux3/4
  [x5] -> Mux3/1
  Fcn7/1 -> [f54y]
  Fcn6/1 -> [f54x]
  [x4] -> Mux3/3
  [y5] -> Mux3/2
  [d45d54] -> Mux3/5
  [f53x] -> Sum3/3
  [f54x] -> Sum3/4
  [f53y] -> Sum4/3
  [f54y] -> Sum4/4
  Constant/1 -> Sum/2
  Sum/1 -> Mux/6
  [h15] -> Sum/1
  Constant1/1 -> Sum1/2
  Sum1/1 -> Mux1/6
  [h25] -> Sum1/1
  Constant2/1 -> Sum2/2
  Sum2/1 -> Mux2/6
  [h35] -> Sum2/1
  Constant3/1 -> Sum5/2
  Sum5/1 -> Mux3/6
  [h45] -> Sum5/1
  [h5oa] -> Sum6/1
  Sum6/1 -> Mux4/6
  Constant4/1 -> Sum6/2
  [d5o1] -> Mux4/5
  [y5] -> Mux4/2
  [x5o1] -> Mux4/3
  Fcn8/1 -> [f5oax]
  Fcn9/1 -> [f5oay]
  [x5] -> Mux4/1
  [y5o1] -> Mux4/4
  Mux4/1 -> Fcn8/1, Fcn9/1
  [f5oax] -> Sum3/5
  [f5oay] -> Sum4/5
  Mux5/1 -> Fcn11/1, Fcn10/1
  [y5o2] -> Mux5/4
  [x5] -> Mux5/1
  Fcn11/1 -> [f5oby]
  Fcn10/1 -> [f5obx]
  [x5o2] -> Mux5/3
  [y5] -> Mux5/2
  [d5o1] -> Mux5/5
  Constant5/1 -> Sum7/2
  Sum7/1 -> Mux5/6
  [h5ob] -> Sum7/1
  [f5obx] -> Sum3/6
  [f5oby] -> Sum4/6

== system Project/Robot 1 /Tracking Control ==
  note: u(6) =th _d
  note: u(5) = error_th
  note: u(4) = derror_y
  note: u(3) = error_y
  note: u(2) = derror_x
  note: u(1) = error_x
  X1 : Inport
  Xd : Inport  Port=2
  Y1 : Inport  Port=3
  Yd : Inport  Port=4
  TH1 : Inport  Port=5
  THc : Inport  Port=6
  Dc : Inport  Port=7
  CC : Inport  Port=8
  CCD : InportShadow  Port=8
  CCTH : InportShadow  Port=8
  Constant : Constant  Value=Dmax
  Derivative2 : Derivative
  Derivative3 : Derivative
  Fcn : Fcn  Expr=K*cos( u(5) )*u(7)
  Fcn1 : Fcn  Expr=K * cos(u(5)) * sin( u(5) + u(6) )*u(7)
  Fcn2 : Fcn  Expr=-K_th*u(5) +u(8)*( u(1)*u(4) - u(3)*u(2) )/( u(1)^2+u(3)^2 )
  Fcn3 : Fcn  Expr=atan2(-u(1),-u(2))
  Fcn4 : Fcn  Expr=(u(1)^2+u(2)^2)*(1/2)
  Fcn5 : Fcn  Expr=cos(u(5)+u(6))
  Integrator1 : Integrator  InitialCondition=init1(2)
  Integrator2 : Integrator  InitialCondition=init1(3)
  Integrator3 : Integrator  InitialCondition=init1(1)
  MinMax : MinMax  Inputs=2  ZeroCross=off
  Mux : Mux  Inputs=8
  Mux1 : Mux  Inputs=2
  Mux2 : Mux  Inputs=2
  Product : Product
  Sum : Sum  Inputs=|-+
  Sum1 : Sum  Inputs=|-+
  Sum2 : Sum  Inputs=|+-
  Sum3 : Sum  Inputs=|+-
  Sum4 : Sum  Inputs=|+-
  Switch : Switch  Criteria=u2 ~= 0  ZeroCross=off
  Switch1 : Switch  Criteria=u2 ~= 0  ZeroCross=off
  Unit Delay : UnitDelay  SampleTime=-1
  Unit Delay1 : UnitDelay  SampleTime=-1
  X : Outport
  Y : Outport  Port=2
  "TH " : Outport  Port=3
  V : Outport  Port=4
  "U " : Outport  Port=5
  wires:
  Integrator1/1 -> Y/1
  Integrator3/1 -> X/1
  Fcn2/1 -> "U "/1, Integrator2/1
  Fcn1/1 -> Sum3/1, Integrator1/1
  Product/1 -> Sum4/1, Integrator3/1
  Fcn5/1 -> Product/2
  Fcn/1 -> Product/1, V/1
  Constant/1 -> MinMax/1
  Integrator2/1 -> "TH "/1
  Mux/1 -> Fcn5/1, Fcn/1, Fcn2/1, Fcn1/1
  Mux1/1 -> Fcn3/1
  Derivative2/1 -> Sum4/2
  Sum2/1 -> Mux/5
  Yd/1 -> [yd], Sum1/1
  Mux2/1 -> Fcn4/1
  [error_y] -> Mux2/2
  Sum/1 -> Mux/1, [error_x]
  [error_x] -> Mux2/1
  Sum3/1 -> [dy1]
  X1/1 -> Sum/2
  TH1/1 -> Sum2/1
  [error_y] -> Mux1/1
  [yd] -> Derivative3/1
  Sum4/1 -> [dx1]
  Derivative3/1 -> Sum3/2
  [error_x] -> Mux1/2
  Sum1/1 -> Mux/3, [error_y]
  Y1/1 -> Sum1/2
  [xd] -> Derivative2/1
  MinMax/1 -> Mux/7
  Xd/1 -> Sum/1, [xd]
  CC/1 -> Mux/8
  Fcn4/1 -> Switch/1
  Dc/1 -> Switch/3
  CCD/1 -> Switch/2
  Switch/1 -> MinMax/2
  Fcn3/1 -> Switch1/1
  THc/1 -> Switch1/3
  Switch1/1 -> Sum2/2, Mux/6
  CCTH/1 -> Switch1/2
  [dx1] -> Unit Delay1/1
  [dy1] -> Unit Delay/1
  Unit Delay1/1 -> Mux/2
  Unit Delay/1 -> Mux/4

== system Project/Robot 2/Tracking Control1 ==
  note: u(6) =th _d
  note: u(5) = error_th
  note: u(4) = derror_y
  note: u(3) = error_y
  note: u(2) = derror_x
  note: u(1) = error_x
  X1 : Inport
  Xd : Inport  Port=2
  Y1 : Inport  Port=3
  Yd : Inport  Port=4
  TH1 : Inport  Port=5
  THc : Inport  Port=6
  Dc : Inport  Port=7
  CC : Inport  Port=8
  CCD : InportShadow  Port=8
  CCTH : InportShadow  Port=8
  Constant : Constant  Value=Dmax
  Derivative2 : Derivative
  Derivative3 : Derivative
  Fcn : Fcn  Expr=K*cos( u(5) )*u(7)
  Fcn1 : Fcn  Expr=K * cos(u(5)) * sin( u(5) + u(6) )*u(7)
  Fcn2 : Fcn  Expr=-K_th*u(5) +u(8)*( u(1)*u(4) - u(3)*u(2) )/( u(1)^2+u(3)^2 )
  Fcn3 : Fcn  Expr=atan2(-u(1),-u(2))
  Fcn4 : Fcn  Expr=(u(1)^2+u(2)^2)*(1/2)
  Fcn5 : Fcn  Expr=cos(u(5)+u(6))
  Integrator1 : Integrator  InitialCondition=init2(2)
  Integrator2 : Integrator  InitialCondition=init2(3)
  Integrator3 : Integrator  InitialCondition=init2(1)
  MinMax : MinMax  Inputs=2
  Mux : Mux  Inputs=8
  Mux1 : Mux  Inputs=2
  Mux2 : Mux  Inputs=2
  Product : Product
  Scope : Scope
  Sum : Sum  Inputs=|-+
  Sum1 : Sum  Inputs=|-+
  Sum2 : Sum  Inputs=|+-
  Sum3 : Sum  Inputs=|+-
  Sum4 : Sum  Inputs=|+-
  Switch : Switch  Criteria=u2 ~= 0
  Switch1 : Switch  Criteria=u2 ~= 0
  Unit Delay : UnitDelay  SampleTime=-1
  Unit Delay1 : UnitDelay  SampleTime=-1
  X : Outport
  Y : Outport  Port=2
  "TH " : Outport  Port=3
  V : Outport  Port=4
  "U " : Outport  Port=5
  wires:
  Integrator1/1 -> Y/1
  Integrator3/1 -> X/1
  Fcn2/1 -> "U "/1, Integrator2/1
  Fcn1/1 -> Sum3/1, Integrator1/1
  Product/1 -> Sum4/1, Integrator3/1
  Fcn5/1 -> Product/2
  Fcn/1 -> Product/1, V/1
  Constant/1 -> MinMax/1
  Integrator2/1 -> "TH "/1
  Mux/1 -> Fcn5/1, Fcn/1, Fcn2/1, Fcn1/1
  Mux1/1 -> Fcn3/1
  Derivative2/1 -> Sum4/2
  Sum2/1 -> Mux/5
  Yd/1 -> [yd], Sum1/1
  Mux2/1 -> Fcn4/1
  [error_y] -> Mux2/2
  Sum/1 -> Mux/1, [error_x]
  [error_x] -> Mux2/1
  Sum3/1 -> [dy1]
  X1/1 -> Sum/2
  TH1/1 -> Sum2/1
  [error_y] -> Mux1/1
  [yd] -> Derivative3/1
  Sum4/1 -> [dx1]
  Derivative3/1 -> Sum3/2
  [error_x] -> Mux1/2
  Sum1/1 -> Mux/3, [error_y]
  Y1/1 -> Sum1/2
  [xd] -> Derivative2/1
  MinMax/1 -> Scope/1, Mux/7
  Xd/1 -> Sum/1, [xd]
  CC/1 -> Mux/8
  Fcn4/1 -> Switch/1
  Dc/1 -> Switch/3
  CCD/1 -> Switch/2
  Switch/1 -> MinMax/2
  Fcn3/1 -> Switch1/1
  THc/1 -> Switch1/3
  Switch1/1 -> Sum2/2, Mux/6
  CCTH/1 -> Switch1/2
  [dx1] -> Unit Delay/1
  [dy1] -> Unit Delay1/1
  Unit Delay/1 -> Mux/2
  Unit Delay1/1 -> Mux/4

== system Project/Robot 3/Tracking Control ==
  note: u(6) =th _d
  note: u(5) = error_th
  note: u(4) = derror_y
  note: u(3) = error_y
  note: u(2) = derror_x
  note: u(1) = error_x
  X1 : Inport
  Xd : Inport  Port=2
  Y1 : Inport  Port=3
  Yd : Inport  Port=4
  TH1 : Inport  Port=5
  THc : Inport  Port=6
  Dc : Inport  Port=7
  CC : Inport  Port=8
  CCD : InportShadow  Port=8
  CCTH : InportShadow  Port=8
  Constant : Constant  Value=Dmax
  Derivative2 : Derivative
  Derivative3 : Derivative
  Fcn : Fcn  Expr=K*cos( u(5) )*u(7)
  Fcn1 : Fcn  Expr=K * cos(u(5)) * sin( u(5) + u(6) )*u(7)
  Fcn2 : Fcn  Expr=-K_th*u(5) +u(8)*( u(1)*u(4) - u(3)*u(2) )/( u(1)^2+u(3)^2 )
  Fcn3 : Fcn  Expr=atan2(-u(1),-u(2))
  Fcn4 : Fcn  Expr=(u(1)^2+u(2)^2)*(1/2)
  Fcn5 : Fcn  Expr=cos(u(5)+u(6))
  Integrator1 : Integrator  InitialCondition=init3(2)
  Integrator2 : Integrator  InitialCondition=init3(3)
  Integrator3 : Integrator  InitialCondition=init3(1)
  MinMax : MinMax  Inputs=2
  Mux : Mux  Inputs=8
  Mux1 : Mux  Inputs=2
  Mux2 : Mux  Inputs=2
  Product : Product
  Scope : Scope
  Sum : Sum  Inputs=|-+
  Sum1 : Sum  Inputs=|-+
  Sum2 : Sum  Inputs=|+-
  Sum3 : Sum  Inputs=|+-
  Sum4 : Sum  Inputs=|+-
  Switch : Switch  Criteria=u2 ~= 0
  Switch1 : Switch  Criteria=u2 ~= 0
  Unit Delay : UnitDelay  SampleTime=-1
  Unit Delay1 : UnitDelay  SampleTime=-1
  X : Outport
  Y : Outport  Port=2
  "TH " : Outport  Port=3
  V : Outport  Port=4
  "U " : Outport  Port=5
  wires:
  Integrator1/1 -> Y/1
  Integrator3/1 -> X/1
  Fcn2/1 -> "U "/1, Integrator2/1
  Fcn1/1 -> Sum3/1, Integrator1/1
  Product/1 -> Sum4/1, Integrator3/1
  Fcn5/1 -> Product/2
  Fcn/1 -> Product/1, V/1
  Constant/1 -> MinMax/1
  Integrator2/1 -> "TH "/1
  Mux/1 -> Fcn5/1, Fcn/1, Fcn2/1, Fcn1/1
  Mux1/1 -> Fcn3/1
  Derivative2/1 -> Sum4/2
  Sum2/1 -> Mux/5
  Yd/1 -> [yd], Sum1/1
  Mux2/1 -> Fcn4/1
  [error_y] -> Mux2/2
  Sum/1 -> Mux/1, [error_x]
  [dy1] -> Unit Delay1/1
  [error_x] -> Mux2/1
  Sum3/1 -> [dy1]
  X1/1 -> Sum/2
  TH1/1 -> Sum2/1
  [error_y] -> Mux1/1
  [yd] -> Derivative3/1
  Sum4/1 -> [dx1]
  Derivative3/1 -> Sum3/2
  [error_x] -> Mux1/2
  Sum1/1 -> Mux/3, [error_y]
  Y1/1 -> Sum1/2
  [xd] -> Derivative2/1
  MinMax/1 -> Scope/1, Mux/7
  Xd/1 -> Sum/1, [xd]
  CC/1 -> Mux/8
  Fcn4/1 -> Switch/1
  Dc/1 -> Switch/3
  CCD/1 -> Switch/2
  Switch/1 -> MinMax/2
  Fcn3/1 -> Switch1/1
  THc/1 -> Switch1/3
  Switch1/1 -> Sum2/2, Mux/6
  CCTH/1 -> Switch1/2
  [dx1] -> Unit Delay/1
  Unit Delay/1 -> Mux/2
  Unit Delay1/1 -> Mux/4
